simulink model "ForwardKinematic_YuMi"  (R2024a)
(part 16 of 23)

Jacobian_right = [(45469976576263333420024314314012801327919322690514472994826407768302665883518778378566397061146074233600072400531729144381613193100703*cos(q1R))/14196068833898572081041480622812588561594557825924180864872855452746861095964803189964668959253194639858643000122386287764347688058880000 + (975695490161691334754993201031873422779992507225204606318647386416514578573291323958060306800265973057287823586614606841372311747139967*sin(q1R))/56784275335594288324165922491250354246378231303696723459491421810987444383859212759858675837012778559434572000489545151057390752235520000 + (27*cos(q5R)*((7514214926474921*sin(q4R)*((9007199067919185*cos(q3R)*((23235800371559029388956996013805*cos(q1R))/40564819207303340847894502572032 - (17274190877287359225804725738355*sin(q1R))/162259276829213363391578010288128))/9007199254740992 + (7514214926474921*cos(q3R)*((7514214926474921*cos(q2R)*((2579692110316253*cos(q1R))/4503599627370496 - (1917820484151683*sin(q1R))/18014398509481984))/36893488147419103232 + sin(q2R)*((1917820484151683*cos(q1R))/18014398509481984 + (2579692110316253*sin(q1R))/4503599627370496)))/36893488147419103232 - sin(q3R)*(cos(q2R)*((1917820484151683*cos(q1R))/18014398509481984 + (2579692110316253*sin(q1R))/4503599627370496) - (7514214926474921*sin(q2R)*((2579692110316253*cos(q1R))/4503599627370496 - (1917820484151683*sin(q1R))/18014398509481984))/36893488147419103232)))/36893488147419103232 + ((9007199067919185*cos(q4R))/9007199254740992 - (234819211581865*sin(q4R))/1152921504606846976)*((129801982932889585091297864435361917839115294955*sin(q1R))/5986310706507378352962293074805895248510699696029696 - (174598797980560374072834504815488878557302284405*cos(q1R))/1496577676626844588240573268701473812127674924007424 + (67682029681889335677290557259385*cos(q2R)*((2579692110316253*cos(q1R))/4503599627370496 - (1917820484151683*sin(q1R))/18014398509481984))/332306998946228968225951765070086144 + (9007199067919185*sin(q2R)*((1917820484151683*cos(q1R))/18014398509481984 + (2579692110316253*sin(q1R))/4503599627370496))/9007199254740992) + ((7514214926474921*cos(q4R))/36893488147419103232 + (4503599440548691*sin(q4R))/4503599627370496)*((9007199067919185*sin(q3R)*((23235800371559029388956996013805*cos(q1R))/40564819207303340847894502572032 - (17274190877287359225804725738355*sin(q1R))/162259276829213363391578010288128))/9007199254740992 + cos(q3R)*(cos(q2R)*((1917820484151683*cos(q1R))/18014398509481984 + (2579692110316253*sin(q1R))/4503599627370496) - (7514214926474921*sin(q2R)*((2579692110316253*cos(q1R))/4503599627370496 - (1917820484151683*sin(q1R))/18014398509481984))/36893488147419103232) + (7514214926474921*sin(q3R)*((7514214926474921*cos(q2R)*((2579692110316253*cos(q1R))/4503599627370496 - (1917820484151683*sin(q1R))/18014398509481984))/36893488147419103232 + sin(q2R)*((1917820484151683*cos(q1R))/18014398509481984 + (2579692110316253*sin(q1R))/4503599627370496)))/36893488147419103232)))/1000 - (202883803014822867*sin(q5R)*((7514214926474921*cos(q4R)*((9007199067919185*cos(q3R)*((23235800371559029388956996013805*cos(q1R))/40564819207303340847894502572032 - (17274190877287359225804725738355*sin(q1R))/162259276829213363391578010288128))/9007199254740992 + (7514214926474921*cos(q3R)*((7514214926474921*cos(q2R)*((2579692110316253*cos(q1R))/4503599627370496 - (1917820484151683*sin(q1R))/18014398509481984))/36893488147419103232 + sin(q2R)*((1917820484151683*cos(q1R))/18014398509481984 + (2579692110316253*sin(q1R))/4503599627370496)))/36893488147419103232 - sin(q3R)*(cos(q2R)*((1917820484151683*cos(q1R))/18014398509481984 + (2579692110316253*sin(q1R))/4503599627370496) - (7514214926474921*sin(q2R)*((2579692110316253*cos(q1R))/4503599627370496 - (1917820484151683*sin(q1R))/18014398509481984))/36893488147419103232)))/36893488147419103232 - ((234819211581865*cos(q4R))/1152921504606846976 + (9007199067919185*sin(q4R))/9007199254740992)*((129801982932889585091297864435361917839115294955*sin(q1R))/5986310706507378352962293074805895248510699696029696 - (174598797980560374072834504815488878557302284405*cos(q1R))/1496577676626844588240573268701473812127674924007424 + (67682029681889335677290557259385*cos(q2R)*((2579692110316253*cos(q1R))/4503599627370496 - (1917820484151683*sin(q1R))/18014398509481984))/332306998946228968225951765070086144 + (9007199067919185*sin(q2R)*((1917820484151683*cos(q1R))/18014398509481984 + (2579692110316253*sin(q1R))/4503599627370496))/9007199254740992) + ((4503599440548691*cos(q4R))/4503599627370496 - (7514214926474921*sin(q4R))/36893488147419103232)*((9007199067919185*sin(q3R)*((23235800371559029388956996013805*cos(q1R))/40564819207303340847894502572032 - (17274190877287359225804725738355*sin(q1R))/162259276829213363391578010288128))/9007199254740992 + cos(q3R)*(cos(q2R)*((1917820484151683*cos(q1R))/18014398509481984 + (2579692110316253*sin(q1R))/4503599627370496) - (7514214926474921*sin(q2R)*((2579692110316253*cos(q1R))/4503599627370496 - (1917820484151683*sin(q1R))/18014398509481984))/36893488147419103232) + (7514214926474921*sin(q3R)*((7514214926474921*cos(q2R)*((2579692110316253*cos(q1R))/4503599627370496 - (1917820484151683*sin(q1R))/18014398509481984))/36893488147419103232 + sin(q2R)*((1917820484151683*cos(q1R))/18014398509481984 + (2579692110316253*sin(q1R))/4503599627370496)))/36893488147419103232)))/36893488147419103232000 - (610321541873521657855151997354401418608858870661075444886782706002880706727*cos(q4R)*((9007199067919185*cos(q3R)*((23235800371559029388956996013805*cos(q1R))/40564819207303340847894502572032 - (17274190877287359225804725738355*sin(q1R))/162259276829213363391578010288128))/9007199254740992 + (7514214926474921*cos(q3R)*((7514214926474921*cos(q2R)*((2579692110316253*cos(q1R))/4503599627370496 - (1917820484151683*sin(q1R))/18014398509481984))/36893488147419103232 + sin(q2R)*((1917820484151683*cos(q1R))/18014398509481984 + (2579692110316253*sin(q1R))/4503599627370496)))/36893488147419103232 - sin(q3R)*(cos(q2R)*((1917820484151683*cos(q1R))/18014398509481984 + (2579692110316253*sin(q1R))/4503599627370496) - (7514214926474921*sin(q2R)*((2579692110316253*cos(q1R))/4503599627370496 - (1917820484151683*sin(q1R))/18014398509481984))/36893488147419103232)))/11307821214581659709333104004754678501295896940003961331978279688272766566400000 - (584133382113593486367040631332731*cos(q6R)*((2056090974134078155817856050893176283501835309672875224633265471054954772650875*cos(q1R))/2085924839766513752338888384931203236916703635113918720651407820138886450957656787131798913024 - (1528559695827542654859482295756575375660057523072748460051910118126597762297125*sin(q1R))/8343699359066055009355553539724812947666814540455674882605631280555545803830627148527195652096 + (67682029681889335677290557259385*cos(q4R)*((9007199067919185*cos(q3R)*((23235800371559029388956996013805*cos(q1R))/40564819207303340847894502572032 - (17274190877287359225804725738355*sin(q1R))/162259276829213363391578010288128))/9007199254740992 + (7514214926474921*cos(q3R)*((7514214926474921*cos(q2R)*((2579692110316253*cos(q1R))/4503599627370496 - (1917820484151683*sin(q1R))/18014398509481984))/36893488147419103232 + sin(q2R)*((1917820484151683*cos(q1R))/18014398509481984 + (2579692110316253*sin(q1R))/4503599627370496)))/36893488147419103232 - sin(q3R)*(cos(q2R)*((1917820484151683*cos(q1R))/18014398509481984 + (2579692110316253*sin(q1R))/4503599627370496) - (7514214926474921*sin(q2R)*((2579692110316253*cos(q1R))/4503599627370496 - (1917820484151683*sin(q1R))/18014398509481984))/36893488147419103232)))/332306998946228968225951765070086144 - (9007199067919185*((234819211581865*cos(q4R))/1152921504606846976 + (9007199067919185*sin(q4R))/9007199254740992)*((129801982932889585091297864435361917839115294955*sin(q1R))/5986310706507378352962293074805895248510699696029696 - (174598797980560374072834504815488878557302284405*cos(q1R))/1496577676626844588240573268701473812127674924007424 + (67682029681889335677290557259385*cos(q2R)*((2579692110316253*cos(q1R))/4503599627370496 - (1917820484151683*sin(q1R))/18014398509481984))/332306998946228968225951765070086144 + (9007199067919185*sin(q2R)*((1917820484151683*cos(q1R))/18014398509481984 + (2579692110316253*sin(q1R))/4503599627370496))/9007199254740992))/9007199254740992 - (609625514665592237562888769449172969868262801225*cos(q3R)*((23235800371559029388956996013805*cos(q1R))/40564819207303340847894502572032 - (17274190877287359225804725738355*sin(q1R))/162259276829213363391578010288128))/2993155353253689176481146537402947624255349848014848 + (15893040848161638993908057577265778144967053025*sin(q3R)*((23235800371559029388956996013805*cos(q1R))/40564819207303340847894502572032 - (17274190877287359225804725738355*sin(q1R))/162259276829213363391578010288128))/383123885216472214589586756787577295904684780545900544 + (9007199067919185*((4503599440548691*cos(q4R))/4503599627370496 - (7514214926474921*sin(q4R))/36893488147419103232)*((9007199067919185*sin(q3R)*((23235800371559029388956996013805*cos(q1R))/40564819207303340847894502572032 - (17274190877287359225804725738355*sin(q1R))/162259276829213363391578010288128))/9007199254740992 + cos(q3R)*(cos(q2R)*((1917820484151683*cos(q1R))/18014398509481984 + (2579692110316253*sin(q1R))/4503599627370496) - (7514214926474921*sin(q2R)*((2579692110316253*cos(q1R))/4503599627370496 - (1917820484151683*sin(q1R))/18014398509481984))/36893488147419103232) + (7514214926474921*sin(q3R)*((7514214926474921*cos(q2R)*((2579692110316253*cos(q1R))/4503599627370496 - (1917820484151683*sin(q1R))/18014398509481984))/36893488147419103232 + sin(q2R)*((1917820484151683*cos(q1R))/18014398509481984 + (2579692110316253*sin(q1R))/4503599627370496)))/36893488147419103232))/9007199254740992 + (1764482024691522628700660907665*cos(q3R)*(cos(q2R)*((1917820484151683*cos(q1R))/18014398509481984 + (2579692110316253*sin(q1R))/4503599627370496) - (7514214926474921*sin(q2R)*((2579692110316253*cos(q1R))/4503599627370496 - (1917820484151683*sin(q1R))/18014398509481984))/36893488147419103232))/42535295865117307932921825928971026432 - (508577317689771495245073589786522929324694383585*cos(q3R)*((7514214926474921*cos(q2R)*((2579692110316253*cos(q1R))/4503599627370496 - (1917820484151683*sin(q1R))/18014398509481984))/36893488147419103232 + sin(q2R)*((1917820484151683*cos(q1R))/18014398509481984 + (2579692110316253*sin(q1R))/4503599627370496)))/12259964326927110866866776217202473468949912977468817408 + (67682029681889335677290557259385*sin(q3R)*(cos(q2R)*((1917820484151683*cos(q1R))/18014398509481984 + (2579692110316253*sin(q1R))/4503599627370496) - (7514214926474921*sin(q2R)*((2579692110316253*cos(q1R))/4503599627370496 - (1917820484151683*sin(q1R))/18014398509481984))/36893488147419103232))/332306998946228968225951765070086144 + (13258697167433729449897784796786197386719169465*sin(q3R)*((7514214926474921*cos(q2R)*((2579692110316253*cos(q1R))/4503599627370496 - (1917820484151683*sin(q1R))/18014398509481984))/36893488147419103232 + sin(q2R)*((1917820484151683*cos(q1R))/18014398509481984 + (2579692110316253*sin(q1R))/4503599627370496)))/1569275433846670190958947355801916604025588861116008628224 - (797029601289130257223357069404502671534492977261568326111352375*cos(q2R)*((2579692110316253*cos(q1R))/4503599627370496 - (1917820484151683*sin(q1R))/18014398509481984))/463168356949264781694283940034751631413079938662562256157830336031652518559744 - (106069577339469832923929692356850887620017617375*sin(q2R)*((1917820484151683*cos(q1R))/18014398509481984 + (2579692110316253*sin(q1R))/4503599627370496))/12554203470773361527671578846415332832204710888928069025792))/16225927682921336339157801028812800 + (94754841554645069948206780163139*sin(q5R)*((7514214926474921*sin(q4R)*((9007199067919185*cos(q3R)*((23235800371559029388956996013805*cos(q1R))/40564819207303340847894502572032 - (17274190877287359225804725738355*sin(q1R))/162259276829213363391578010288128))/9007199254740992 + (7514214926474921*cos(q3R)*((7514214926474921*cos(q2R)*((2579692110316253*cos(q1R))/4503599627370496 - (1917820484151683*sin(q1R))/18014398509481984))/36893488147419103232 + sin(q2R)*((1917820484151683*cos(q1R))/18014398509481984 + (2579692110316253*sin(q1R))/4503599627370496)))/36893488147419103232 - sin(q3R)*(cos(q2R)*((1917820484151683*cos(q1R))/18014398509481984 + (2579692110316253*sin(q1R))/4503599627370496) - (7514214926474921*sin(q2R)*((2579692110316253*cos(q1R))/4503599627370496 - (1917820484151683*sin(q1R))/18014398509481984))/36893488147419103232)))/36893488147419103232 + ((9007199067919185*cos(q4R))/9007199254740992 - (234819211581865*sin(q4R))/1152921504606846976)*((129801982932889585091297864435361917839115294955*sin(q1R))/5986310706507378352962293074805895248510699696029696 - (174598797980560374072834504815488878557302284405*cos(q1R))/1496577676626844588240573268701473812127674924007424 + (67682029681889335677290557259385*cos(q2R)*((2579692110316253*cos(q1R))/4503599627370496 - (1917820484151683*sin(q1R))/18014398509481984))/332306998946228968225951765070086144 + (9007199067919185*sin(q2R)*((1917820484151683*cos(q1R))/18014398509481984 + (2579692110316253*sin(q1R))/4503599627370496))/9007199254740992) + ((7514214926474921*cos(q4R))/36893488147419103232 + (4503599440548691*sin(q4R))/4503599627370496)*((9007199067919185*sin(q3R)*((23235800371559029388956996013805*cos(q1R))/40564819207303340847894502572032 - (17274190877287359225804725738355*sin(q1R))/162259276829213363391578010288128))/9007199254740992 + cos(q3R)*(cos(q2R)*((1917820484151683*cos(q1R))/18014398509481984 + (2579692110316253*sin(q1R))/4503599627370496) - (7514214926474921*sin(q2R)*((2579692110316253*cos(q1R))/4503599627370496 - (1917820484151683*sin(q1R))/18014398509481984))/36893488147419103232) + (7514214926474921*sin(q3R)*((7514214926474921*cos(q2R)*((2579692110316253*cos(q1R))/4503599627370496 - (1917820484151683*sin(q1R))/18014398509481984))/36893488147419103232 + sin(q2R)*((1917820484151683*cos(q1R))/18014398509481984 + (2579692110316253*sin(q1R))/4503599627370496)))/36893488147419103232)))/66461399789245793645190353014017228800 - (608651409044468601*sin(q4R)*((9007199067919185*cos(q3R)*((23235800371559029388956996013805*cos(q1R))/40564819207303340847894502572032 - (17274190877287359225804725738355*sin(q1R))/162259276829213363391578010288128))/9007199254740992 + (7514214926474921*cos(q3R)*((7514214926474921*cos(q2R)*((2579692110316253*cos(q1R))/4503599627370496 - (1917820484151683*sin(q1R))/18014398509481984))/36893488147419103232 + sin(q2R)*((1917820484151683*cos(q1R))/18014398509481984 + (2579692110316253*sin(q1R))/4503599627370496)))/36893488147419103232 - sin(q3R)*(cos(q2R)*((1917820484151683*cos(q1R))/18014398509481984 + (2579692110316253*sin(q1R))/4503599627370496) - (7514214926474921*sin(q2R)*((2579692110316253*cos(q1R))/4503599627370496 - (1917820484151683*sin(q1R))/18014398509481984))/36893488147419103232)))/73786976294838206464000 - (48638874966763599*sin(q6R)*((2056090974134078155817856050893176283501835309672875224633265471054954772650875*cos(q1R))/2085924839766513752338888384931203236916703635113918720651407820138886450957656787131798913024 - (1528559695827542654859482295756575375660057523072748460051910118126597762297125*sin(q1R))/8343699359066055009355553539724812947666814540455674882605631280555545803830627148527195652096 + (67682029681889335677290557259385*cos(q4R)*((9007199067919185*cos(q3R)*((23235800371559029388956996013805*cos(q1R))/40564819207303340847894502572032 - (17274190877287359225804725738355*sin(q1R))/162259276829213363391578010288128))/9007199254740992 + (7514214926474921*cos(q3R)*((7514214926474921*cos(q2R)*((2579692110316253*cos(q1R))/4503599627370496 - (1917820484151683*sin(q1R))/18014398509481984))/36893488147419103232 + sin(q2R)*((1917820484151683*cos(q1R))/18014398509481984 + (2579692110316253*sin(q1R))/4503599627370496)))/36893488147419103232 - sin(q3R)*(cos(q2R)*((1917820484151683*cos(q1R))/18014398509481984 + (2579692110316253*sin(q1R))/4503599627370496) - (7514214926474921*sin(q2R)*((2579692110316253*cos(q1R))/4503599627370496 - (1917820484151683*sin(q1R))/18014398509481984))/36893488147419103232)))/332306998946228968225951765070086144 - (9007199067919185*((234819211581865*cos(q4R))/1152921504606846976 + (9007199067919185*sin(q4R))/9007199254740992)*((129801982932889585091297864435361917839115294955*sin(q1R))/5986310706507378352962293074805895248510699696029696 - (174598797980560374072834504815488878557302284405*cos(q1R))/1496577676626844588240573268701473812127674924007424 + (67682029681889335677290557259385*cos(q2R)*((2579692110316253*cos(q1R))/4503599627370496 - (1917820484151683*sin(q1R))/18014398509481984))/332306998946228968225951765070086144 + (9007199067919185*sin(q2R)*((1917820484151683*cos(q1R))/18014398509481984 + (2579692110316253*sin(q1R))/4503599627370496))/9007199254740992))/9007199254740992 - (609625514665592237562888769449172969868262801225*cos(q3R)*((23235800371559029388956996013805*cos(q1R))/40564819207303340847894502572032 - (17274190877287359225804725738355*sin(q1R))/162259276829213363391578010288128))/2993155353253689176481146537402947624255349848014848 + (15893040848161638993908057577265778144967053025*sin(q3R)*((23235800371559029388956996013805*cos(q1R))/40564819207303340847894502572032 - (17274190877287359225804725738355*sin(q1R))/162259276829213363391578010288128))/383123885216472214589586756787577295904684780545900544 + (9007199067919185*((4503599440548691*cos(q4R))/4503599627370496 - (7514214926474921*sin(q4R))/36893488147419103232)*((9007199067919185*sin(q3R)*((23235800371559029388956996013805*cos(q1R))/40564819207303340847894502572032 - (17274190877287359225804725738355*sin(q1R))/162259276829213363391578010288128))/9007199254740992 + cos(q3R)*(cos(q2R)*((1917820484151683*cos(q1R))/18014398509481984 + (2579692110316253*sin(q1R))/4503599627370496) - (7514214926474921*sin(q2R)*((2579692110316253*cos(q1R))/4503599627370496 - (1917820484151683*sin(q1R))/18014398509481984))/36893488147419103232) + (7514214926474921*sin(q3R)*((7514214926474921*cos(q2R)*((2579692110316253*cos(q1R))/4503599627370496 - (1917820484151683*sin(q1R))/18014398509481984))/36893488147419103232 + sin(q2R)*((1917820484151683*cos(q1R))/18014398509481984 + (2579692110316253*sin(q1R))/4503599627370496)))/36893488147419103232))/9007199254740992 + (1764482024691522628700660907665*cos(q3R)*(cos(q2R)*((1917820484151683*cos(q1R))/18014398509481984 + (2579692110316253*sin(q1R))/4503599627370496) - (7514214926474921*sin(q2R)*((2579692110316253*cos(q1R))/4503599627370496 - (1917820484151683*sin(q1R))/18014398509481984))/36893488147419103232))/42535295865117307932921825928971026432 - (508577317689771495245073589786522929324694383585*cos(q3R)*((7514214926474921*cos(q2R)*((2579692110316253*cos(q1R))/4503599627370496 - (1917820484151683*sin(q1R))/18014398509481984))/36893488147419103232 + sin(q2R)*((1917820484151683*cos(q1R))/18014398509481984 + (2579692110316253*sin(q1R))/4503599627370496)))/12259964326927110866866776217202473468949912977468817408 + (67682029681889335677290557259385*sin(q3R)*(cos(q2R)*((1917820484151683*cos(q1R))/18014398509481984 + (2579692110316253*sin(q1R))/4503599627370496) - (7514214926474921*sin(q2R)*((2579692110316253*cos(q1R))/4503599627370496 - (1917820484151683*sin(q1R))/18014398509481984))/36893488147419103232))/332306998946228968225951765070086144 + (13258697167433729449897784796786197386719169465*sin(q3R)*((7514214926474921*cos(q2R)*((2579692110316253*cos(q1R))/4503599627370496 - (1917820484151683*sin(q1R))/18014398509481984))/36893488147419103232 + sin(q2R)*((1917820484151683*cos(q1R))/18014398509481984 + (2579692110316253*sin(q1R))/4503599627370496)))/1569275433846670190958947355801916604025588861116008628224 - (797029601289130257223357069404502671534492977261568326111352375*cos(q2R)*((2579692110316253*cos(q1R))/4503599627370496 - (1917820484151683*sin(q1R))/18014398509481984))/463168356949264781694283940034751631413079938662562256157830336031652518559744 - (106069577339469832923929692356850887620017617375*sin(q2R)*((1917820484151683*cos(q1R))/18014398509481984 + (2579692110316253*sin(q1R))/4503599627370496))/12554203470773361527671578846415332832204710888928069025792))/1801439850948198400 - (81*((9007199067919185*cos(q4R))/9007199254740992 - (234819211581865*sin(q4R))/1152921504606846976)*((129801982932889585091297864435361917839115294955*sin(q1R))/5986310706507378352962293074805895248510699696029696 - (174598797980560374072834504815488878557302284405*cos(q1R))/1496577676626844588240573268701473812127674924007424 + (67682029681889335677290557259385*cos(q2R)*((2579692110316253*cos(q1R))/4503599627370496 - (1917820484151683*sin(q1R))/18014398509481984))/332306998946228968225951765070086144 + (9007199067919185*sin(q2R)*((1917820484151683*cos(q1R))/18014398509481984 + (2579692110316253*sin(q1R))/4503599627370496))/9007199254740992))/2000 + (81222263116692158804177042061221826384594597321566869716687*((234819211581865*cos(q4R))/1152921504606846976 + (9007199067919185*sin(q4R))/9007199254740992)*((129801982932889585091297864435361917839115294955*sin(q1R))/5986310706507378352962293074805895248510699696029696 - (174598797980560374072834504815488878557302284405*cos(q1R))/1496577676626844588240573268701473812127674924007424 + (67682029681889335677290557259385*cos(q2R)*((2579692110316253*cos(q1R))/4503599627370496 - (1917820484151683*sin(q1R))/18014398509481984))/332306998946228968225951765070086144 + (9007199067919185*sin(q2R)*((1917820484151683*cos(q1R))/18014398509481984 + (2579692110316253*sin(q1R))/4503599627370496))/9007199254740992))/306499108173177771671669405430061836723747824436720435200000 - (170695144106365826517608855445768431563113584343*cos(q5R)*((273626851807209941619219010639387076236787289365779842797695875*cos(q1R))/56539106072908298546665520023773392506479484700019806659891398441363832832 - (203422408166946418981152780445187297537016008229516441756292125*sin(q1R))/226156424291633194186662080095093570025917938800079226639565593765455331328 - (81129635049124235038645691064225*cos(q3R)*((23235800371559029388956996013805*cos(q1R))/40564819207303340847894502572032 - (17274190877287359225804725738355*sin(q1R))/162259276829213363391578010288128))/81129638414606681695789005144064 + (2115063383689692319117831580025*sin(q3R)*((23235800371559029388956996013805*cos(q1R))/40564819207303340847894502572032 - (17274190877287359225804725738355*sin(q1R))/162259276829213363391578010288128))/10384593717069655257060992658440192 + (234819211581865*cos(q3R)*(cos(q2R)*((1917820484151683*cos(q1R))/18014398509481984 + (2579692110316253*sin(q1R))/4503599627370496) - (7514214926474921*sin(q2R)*((2579692110316253*cos(q1R))/4503599627370496 - (1917820484151683*sin(q1R))/18014398509481984))/36893488147419103232))/1152921504606846976 - (67682029681889335677290557259385*cos(q3R)*((7514214926474921*cos(q2R)*((2579692110316253*cos(q1R))/4503599627370496 - (1917820484151683*sin(q1R))/18014398509481984))/36893488147419103232 + sin(q2R)*((1917820484151683*cos(q1R))/18014398509481984 + (2579692110316253*sin(q1R))/4503599627370496)))/332306998946228968225951765070086144 + (9007199067919185*sin(q3R)*(cos(q2R)*((1917820484151683*cos(q1R))/18014398509481984 + (2579692110316253*sin(q1R))/4503599627370496) - (7514214926474921*sin(q2R)*((2579692110316253*cos(q1R))/4503599627370496 - (1917820484151683*sin(q1R))/18014398509481984))/36893488147419103232))/9007199254740992 + (1764482024691522628700660907665*sin(q3R)*((7514214926474921*cos(q2R)*((2579692110316253*cos(q1R))/4503599627370496 - (1917820484151683*sin(q1R))/18014398509481984))/36893488147419103232 + sin(q2R)*((1917820484151683*cos(q1R))/18014398509481984 + (2579692110316253*sin(q1R))/4503599627370496)))/42535295865117307932921825928971026432 - (106069577339469832923929692356850887620017617375*cos(q2R)*((2579692110316253*cos(q1R))/4503599627370496 - (1917820484151683*sin(q1R))/18014398509481984))/12554203470773361527671578846415332832204710888928069025792 - (14115856197532180673579726082375*sin(q2R)*((1917820484151683*cos(q1R))/18014398509481984 + (2579692110316253*sin(q1R))/4503599627370496))/340282366920938463463374607431768211456))/119726214130147567059245861496117904970213993920593920 + (48638874966763599*sin(q5R)*((273626851807209941619219010639387076236787289365779842797695875*cos(q1R))/56539106072908298546665520023773392506479484700019806659891398441363832832 - (203422408166946418981152780445187297537016008229516441756292125*sin(q1R))/226156424291633194186662080095093570025917938800079226639565593765455331328 - (81129635049124235038645691064225*cos(q3R)*((23235800371559029388956996013805*cos(q1R))/40564819207303340847894502572032 - (17274190877287359225804725738355*sin(q1R))/162259276829213363391578010288128))/81129638414606681695789005144064 + (2115063383689692319117831580025*sin(q3R)*((23235800371559029388956996013805*cos(q1R))/40564819207303340847894502572032 - (17274190877287359225804725738355*sin(q1R))/162259276829213363391578010288128))/10384593717069655257060992658440192 + (234819211581865*cos(q3R)*(cos(q2R)*((1917820484151683*cos(q1R))/18014398509481984 + (2579692110316253*sin(q1R))/4503599627370496) - (7514214926474921*sin(q2R)*((2579692110316253*cos(q1R))/4503599627370496 - (1917820484151683*sin(q1R))/18014398509481984))/36893488147419103232))/1152921504606846976 - (67682029681889335677290557259385*cos(q3R)*((7514214926474921*cos(q2R)*((2579692110316253*cos(q1R))/4503599627370496 - (1917820484151683*sin(q1R))/18014398509481984))/36893488147419103232 + sin(q2R)*((1917820484151683*cos(q1R))/18014398509481984 + (2579692110316253*sin(q1R))/4503599627370496)))/332306998946228968225951765070086144 + (9007199067919185*sin(q3R)*(cos(q2R)*((1917820484151683*cos(q1R))/18014398509481984 + (2579692110316253*sin(q1R))/4503599627370496) - (7514214926474921*sin(q2R)*((2579692110316253*cos(q1R))/4503599627370496 - (1917820484151683*sin(q1R))/18014398509481984))/36893488147419103232))/9007199254740992 + (1764482024691522628700660907665*sin(q3R)*((7514214926474921*cos(q2R)*((2579692110316253*cos(q1R))/4503599627370496 - (1917820484151683*sin(q1R))/18014398509481984))/36893488147419103232 + sin(q2R)*((1917820484151683*cos(q1R))/18014398509481984 + (2579692110316253*sin(q1R))/4503599627370496)))/42535295865117307932921825928971026432 - (106069577339469832923929692356850887620017617375*cos(q2R)*((2579692110316253*cos(q1R))/4503599627370496 - (1917820484151683*sin(q1R))/18014398509481984))/12554203470773361527671578846415332832204710888928069025792 - (14115856197532180673579726082375*sin(q2R)*((1917820484151683*cos(q1R))/18014398509481984 + (2579692110316253*sin(q1R))/4503599627370496))/340282366920938463463374607431768211456))/1801439850948198400 - (2436553109258773196144549622003023*cos(q6R)*(sin(q5R)*((7514214926474921*sin(q4R)*((9007199067919185*cos(q3R)*((23235800371559029388956996013805*cos(q1R))/40564819207303340847894502572032 - (17274190877287359225804725738355*sin(q1R))/162259276829213363391578010288128))/9007199254740992 + (7514214926474921*cos(q3R)*((7514214926474921*cos(q2R)*((2579692110316253*cos(q1R))/4503599627370496 - (1917820484151683*sin(q1R))/18014398509481984))/36893488147419103232 + sin(q2R)*((1917820484151683*cos(q1R))/18014398509481984 + (2579692110316253*sin(q1R))/4503599627370496)))/36893488147419103232 - sin(q3R)*(cos(q2R)*((1917820484151683*cos(q1R))/18014398509481984 + (2579692110316253*sin(q1R))/4503599627370496) - (7514214926474921*sin(q2R)*((2579692110316253*cos(q1R))/4503599627370496 - (1917820484151683*sin(q1R))/18014398509481984))/36893488147419103232)))/36893488147419103232 + ((9007199067919185*cos(q4R))/9007199254740992 - (234819211581865*sin(q4R))/1152921504606846976)*((129801982932889585091297864435361917839115294955*sin(q1R))/5986310706507378352962293074805895248510699696029696 - (174598797980560374072834504815488878557302284405*cos(q1R))/1496577676626844588240573268701473812127674924007424 + (67682029681889335677290557259385*cos(q2R)*((2579692110316253*cos(q1R))/4503599627370496 - (1917820484151683*sin(q1R))/18014398509481984))/332306998946228968225951765070086144 + (9007199067919185*sin(q2R)*((1917820484151683*cos(q1R))/18014398509481984 + (2579692110316253*sin(q1R))/4503599627370496))/9007199254740992) + ((7514214926474921*cos(q4R))/36893488147419103232 + (4503599440548691*sin(q4R))/4503599627370496)*((9007199067919185*sin(q3R)*((23235800371559029388956996013805*cos(q1R))/40564819207303340847894502572032 - (17274190877287359225804725738355*sin(q1R))/162259276829213363391578010288128))/9007199254740992 + cos(q3R)*(cos(q2R)*((1917820484151683*cos(q1R))/18014398509481984 + (2579692110316253*sin(q1R))/4503599627370496) - (7514214926474921*sin(q2R)*((2579692110316253*cos(q1R))/4503599627370496 - (1917820484151683*sin(q1R))/18014398509481984))/36893488147419103232) + (7514214926474921*sin(q3R)*((7514214926474921*cos(q2R)*((2579692110316253*cos(q1R))/4503599627370496 - (1917820484151683*sin(q1R))/18014398509481984))/36893488147419103232 + sin(q2R)*((1917820484151683*cos(q1R))/18014398509481984 + (2579692110316253*sin(q1R))/4503599627370496)))/36893488147419103232)) - (9007199067919185*cos(q5R)*((273626851807209941619219010639387076236787289365779842797695875*cos(q1R))/56539106072908298546665520023773392506479484700019806659891398441363832832 - (203422408166946418981152780445187297537016008229516441756292125*sin(q1R))/226156424291633194186662080095093570025917938800079226639565593765455331328 - (81129635049124235038645691064225*cos(q3R)*((23235800371559029388956996013805*cos(q1R))/40564819207303340847894502572032 - (17274190877287359225804725738355*sin(q1R))/162259276829213363391578010288128))/81129638414606681695789005144064 + (2115063383689692319117831580025*sin(q3R)*((23235800371559029388956996013805*cos(q1R))/40564819207303340847894502572032 - (17274190877287359225804725738355*sin(q1R))/162259276829213363391578010288128))/10384593717069655257060992658440192 + (234819211581865*cos(q3R)*(cos(q2R)*((1917820484151683*cos(q1R))/18014398509481984 + (2579692110316253*sin(q1R))/4503599627370496) - (7514214926474921*sin(q2R)*((2579692110316253*cos(q1R))/4503599627370496 - (1917820484151683*sin(q1R))/18014398509481984))/36893488147419103232))/1152921504606846976 - (67682029681889335677290557259385*cos(q3R)*((7514214926474921*cos(q2R)*((2579692110316253*cos(q1R))/4503599627370496 - (1917820484151683*sin(q1R))/18014398509481984))/36893488147419103232 + sin(q2R)*((1917820484151683*cos(q1R))/18014398509481984 + (2579692110316253*sin(q1R))/4503599627370496)))/332306998946228968225951765070086144 + (9007199067919185*sin(q3R)*(cos(q2R)*((1917820484151683*cos(q1R))/18014398509481984 + (2579692110316253*sin(q1R))/4503599627370496) - (7514214926474921*sin(q2R)*((2579692110316253*cos(q1R))/4503599627370496 - (1917820484151683*sin(q1R))/18014398509481984))/36893488147419103232))/9007199254740992 + (1764482024691522628700660907665*sin(q3R)*((7514214926474921*cos(q2R)*((2579692110316253*cos(q1R))/4503599627370496 - (1917820484151683*sin(q1R))/18014398509481984))/36893488147419103232 + sin(q2R)*((1917820484151683*cos(q1R))/18014398509481984 + (2579692110316253*sin(q1R))/4503599627370496)))/42535295865117307932921825928971026432 - (106069577339469832923929692356850887620017617375*cos(q2R)*((2579692110316253*cos(q1R))/4503599627370496 - (1917820484151683*sin(q1R))/18014398509481984))/12554203470773361527671578846415332832204710888928069025792 - (14115856197532180673579726082375*sin(q2R)*((1917820484151683*cos(q1R))/18014398509481984 + (2579692110316253*sin(q1R))/4503599627370496))/340282366920938463463374607431768211456))/9007199254740992 + (7514214926474921*cos(q5R)*((7514214926474921*cos(q4R)*((9007199067919185*cos(q3R)*((23235800371559029388956996013805*cos(q1R))/40564819207303340847894502572032 - (17274190877287359225804725738355*sin(q1R))/162259276829213363391578010288128))/9007199254740992 + (7514214926474921*cos(q3R)*((7514214926474921*cos(q2R)*((2579692110316253*cos(q1R))/4503599627370496 - (1917820484151683*sin(q1R))/18014398509481984))/36893488147419103232 + sin(q2R)*((1917820484151683*cos(q1R))/18014398509481984 + (2579692110316253*sin(q1R))/4503599627370496)))/36893488147419103232 - sin(q3R)*(cos(q2R)*((1917820484151683*cos(q1R))/18014398509481984 + (2579692110316253*sin(q1R))/4503599627370496) - (7514214926474921*sin(q2R)*((2579692110316253*cos(q1R))/4503599627370496 - (1917820484151683*sin(q1R))/18014398509481984))/36893488147419103232)))/36893488147419103232 - ((234819211581865*cos(q4R))/1152921504606846976 + (9007199067919185*sin(q4R))/9007199254740992)*((129801982932889585091297864435361917839115294955*sin(q1R))/5986310706507378352962293074805895248510699696029696 - (174598797980560374072834504815488878557302284405*cos(q1R))/1496577676626844588240573268701473812127674924007424 + (67682029681889335677290557259385*cos(q2R)*((2579692110316253*cos(q1R))/4503599627370496 - (1917820484151683*sin(q1R))/18014398509481984))/332306998946228968225951765070086144 + (9007199067919185*sin(q2R)*((1917820484151683*cos(q1R))/18014398509481984 + (2579692110316253*sin(q1R))/4503599627370496))/9007199254740992) + ((4503599440548691*cos(q4R))/4503599627370496 - (7514214926474921*sin(q4R))/36893488147419103232)*((9007199067919185*sin(q3R)*((23235800371559029388956996013805*cos(q1R))/40564819207303340847894502572032 - (17274190877287359225804725738355*sin(q1R))/162259276829213363391578010288128))/9007199254740992 + cos(q3R)*(cos(q2R)*((1917820484151683*cos(q1R))/18014398509481984 + (2579692110316253*sin(q1R))/4503599627370496) - (7514214926474921*sin(q2R)*((2579692110316253*cos(q1R))/4503599627370496 - (1917820484151683*sin(q1R))/18014398509481984))/36893488147419103232) + (7514214926474921*sin(q3R)*((7514214926474921*cos(q2R)*((2579692110316253*cos(q1R))/4503599627370496 - (1917820484151683*sin(q1R))/18014398509481984))/36893488147419103232 + sin(q2R)*((1917820484151683*cos(q1R))/18014398509481984 + (2579692110316253*sin(q1R))/4503599627370496)))/36893488147419103232)))/36893488147419103232))/332306998946228968225951765070086144000 - (27*cos(q6R)*(cos(q5R)*((7514214926474921*sin(q4R)*((9007199067919185*cos(q3R)*((23235800371559029388956996013805*cos(q1R))/40564819207303340847894502572032 - (17274190877287359225804725738355*sin(q1R))/162259276829213363391578010288128))/9007199254740992 + (7514214926474921*cos(q3R)*((7514214926474921*cos(q2R)*((2579692110316253*cos(q1R))/4503599627370496 - (1917820484151683*sin(q1R))/18014398509481984))/36893488147419103232 + sin(q2R)*((1917820484151683*cos(q1R))/18014398509481984 + (2579692110316253*sin(q1R))/4503599627370496)))/36893488147419103232 - sin(q3R)*(cos(q2R)*((1917820484151683*cos(q1R))/18014398509481984 + (2579692110316253*sin(q1R))/4503599627370496) - (7514214926474921*sin(q2R)*((2579692110316253*cos(q1R))/4503599627370496 - (1917820484151683*sin(q1R))/18014398509481984))/36893488147419103232)))/36893488147419103232 + ((9007199067919185*cos(q4R))/9007199254740992 - (234819211581865*sin(q4R))/1152921504606846976)*((129801982932889585091297864435361917839115294955*sin(q1R))/5986310706507378352962293074805895248510699696029696 - (174598797980560374072834504815488878557302284405*cos(q1R))/1496577676626844588240573268701473812127674924007424 + (67682029681889335677290557259385*cos(q2R)*((2579692110316253*cos(q1R))/4503599627370496 - (1917820484151683*sin(q1R))/18014398509481984))/332306998946228968225951765070086144 + (9007199067919185*sin(q2R)*((1917820484151683*cos(q1R))/18014398509481984 + (2579692110316253*sin(q1R))/4503599627370496))/9007199254740992) + ((7514214926474921*cos(q4R))/36893488147419103232 + (4503599440548691*sin(q4R))/4503599627370496)*((9007199067919185*sin(q3R)*((23235800371559029388956996013805*cos(q1R))/40564819207303340847894502572032 - (17274190877287359225804725738355*sin(q1R))/162259276829213363391578010288128))/9007199254740992 + cos(q3R)*(cos(q2R)*((1917820484151683*cos(q1R))/18014398509481984 + (2579692110316253*sin(q1R))/4503599627370496) - (7514214926474921*sin(q2R)*((2579692110316253*cos(q1R))/4503599627370496 - (1917820484151683*sin(q1R))/18014398509481984))/36893488147419103232) + (7514214926474921*sin(q3R)*((7514214926474921*cos(q2R)*((2579692110316253*cos(q1R))/4503599627370496 - (1917820484151683*sin(q1R))/18014398509481984))/36893488147419103232 + sin(q2R)*((1917820484151683*cos(q1R))/18014398509481984 + (2579692110316253*sin(q1R))/4503599627370496)))/36893488147419103232)) - (7514214926474921*sin(q5R)*((7514214926474921*cos(q4R)*((9007199067919185*cos(q3R)*((23235800371559029388956996013805*cos(q1R))/40564819207303340847894502572032 - (17274190877287359225804725738355*sin(q1R))/162259276829213363391578010288128))/9007199254740992 + (7514214926474921*cos(q3R)*((7514214926474921*cos(q2R)*((2579692110316253*cos(q1R))/4503599627370496 - (1917820484151683*sin(q1R))/18014398509481984))/36893488147419103232 + sin(q2R)*((1917820484151683*cos(q1R))/18014398509481984 + (2579692110316253*sin(q1R))/4503599627370496)))/36893488147419103232 - sin(q3R)*(cos(q2R)*((1917820484151683*cos(q1R))/18014398509481984 + (2579692110316253*sin(q1R))/4503599627370496) - (7514214926474921*sin(q2R)*((2579692110316253*cos(q1R))/4503599627370496 - (1917820484151683*sin(q1R))/18014398509481984))/36893488147419103232)))/36893488147419103232 - ((234819211581865*cos(q4R))/1152921504606846976 + (9007199067919185*sin(q4R))/9007199254740992)*((129801982932889585091297864435361917839115294955*sin(q1R))/5986310706507378352962293074805895248510699696029696 - (174598797980560374072834504815488878557302284405*cos(q1R))/1496577676626844588240573268701473812127674924007424 + (67682029681889335677290557259385*cos(q2R)*((2579692110316253*cos(q1R))/4503599627370496 - (1917820484151683*sin(q1R))/18014398509481984))/332306998946228968225951765070086144 + (9007199067919185*sin(q2R)*((1917820484151683*cos(q1R))/18014398509481984 + (2579692110316253*sin(q1R))/4503599627370496))/9007199254740992) + ((4503599440548691*cos(q4R))/4503599627370496 - (7514214926474921*sin(q4R))/36893488147419103232)*((9007199067919185*sin(q3R)*((23235800371559029388956996013805*cos(q1R))/40564819207303340847894502572032 - (17274190877287359225804725738355*sin(q1R))/162259276829213363391578010288128))/9007199254740992 + cos(q3R)*(cos(q2R)*((1917820484151683*cos(q1R))/18014398509481984 + (2579692110316253*sin(q1R))/4503599627370496) - (7514214926474921*sin(q2R)*((2579692110316253*cos(q1R))/4503599627370496 - (1917820484151683*sin(q1R))/18014398509481984))/36893488147419103232) + (7514214926474921*sin(q3R)*((7514214926474921*cos(q2R)*((2579692110316253*cos(q1R))/4503599627370496 - (1917820484151683*sin(q1R))/18014398509481984))/36893488147419103232 + sin(q2R)*((1917820484151683*cos(q1R))/18014398509481984 + (2579692110316253*sin(q1R))/4503599627370496)))/36893488147419103232)))/36893488147419103232 + (9007199067919185*sin(q5R)*((273626851807209941619219010639387076236787289365779842797695875*cos(q1R))/56539106072908298546665520023773392506479484700019806659891398441363832832 - (203422408166946418981152780445187297537016008229516441756292125*sin(q1R))/226156424291633194186662080095093570025917938800079226639565593765455331328 - (81129635049124235038645691064225*cos(q3R)*((23235800371559029388956996013805*cos(q1R))/40564819207303340847894502572032 - (17274190877287359225804725738355*sin(q1R))/162259276829213363391578010288128))/81129638414606681695789005144064 + (2115063383689692319117831580025*sin(q3R)*((23235800371559029388956996013805*cos(q1R))/40564819207303340847894502572032 - (17274190877287359225804725738355*sin(q1R))/162259276829213363391578010288128))/10384593717069655257060992658440192 + (234819211581865*cos(q3R)*(cos(q2R)*((1917820484151683*cos(q1R))/18014398509481984 + (2579692110316253*sin(q1R))/4503599627370496) - (7514214926474921*sin(q2R)*((2579692110316253*cos(q1R))/4503599627370496 - (1917820484151683*sin(q1R))/18014398509481984))/36893488147419103232))/1152921504606846976 - (67682029681889335677290557259385*cos(q3R)*((7514214926474921*cos(q2R)*((2579692110316253*cos(q1R))/4503599627370496 - (1917820484151683*sin(q1R))/18014398509481984))/36893488147419103232 + sin(q2R)*((1917820484151683*cos(q1R))/18014398509481984 + (2579692110316253*sin(q1R))/4503599627370496)))/332306998946228968225951765070086144 + (9007199067919185*sin(q3R)*(cos(q2R)*((1917820484151683*cos(q1R))/18014398509481984 + (2579692110316253*sin(q1R))/4503599627370496) - (7514214926474921*sin(q2R)*((2579692110316253*cos(q1R))/4503599627370496 - (1917820484151683*sin(q1R))/18014398509481984))/36893488147419103232))/9007199254740992 + (1764482024691522628700660907665*sin(q3R)*((7514214926474921*cos(q2R)*((2579692110316253*cos(q1R))/4503599627370496 - (1917820484151683*sin(q1R))/18014398509481984))/36893488147419103232 + sin(q2R)*((1917820484151683*cos(q1R))/18014398509481984 + (2579692110316253*sin(q1R))/4503599627370496)))/42535295865117307932921825928971026432 - (106069577339469832923929692356850887620017617375*cos(q2R)*((2579692110316253*cos(q1R))/4503599627370496 - (1917820484151683*sin(q1R))/18014398509481984))/12554203470773361527671578846415332832204710888928069025792 - (14115856197532180673579726082375*sin(q2R)*((1917820484151683*cos(q1R))/18014398509481984 + (2579692110316253*sin(q1R))/4503599627370496))/340282366920938463463374607431768211456))/9007199254740992))/1000 - (202883803014822867*sin(q6R)*(sin(q5R)*((7514214926474921*sin(q4R)*((9007199067919185*cos(q3R)*((23235800371559029388956996013805*cos(q1R))/40564819207303340847894502572032 - (17274190877287359225804725738355*sin(q1R))/162259276829213363391578010288128))/9007199254740992 + (7514214926474921*cos(q3R)*((7514214926474921*cos(q2R)*((2579692110316253*cos(q1R))/4503599627370496 - (1917820484151683*sin(q1R))/18014398509481984))/36893488147419103232 + sin(q2R)*((1917820484151683*cos(q1R))/18014398509481984 + (2579692110316253*sin(q1R))/4503599627370496)))/36893488147419103232 - sin(q3R)*(cos(q2R)*((1917820484151683*cos(q1R))/18014398509481984 + (2579692110316253*sin(q1R))/4503599627370496) - (7514214926474921*sin(q2R)*((2579692110316253*cos(q1R))/4503599627370496 - (1917820484151683*sin(q1R))/18014398509481984))/36893488147419103232)))/36893488147419103232 + ((9007199067919185*cos(q4R))/9007199254740992 - (234819211581865*sin(q4R))/1152921504606846976)*((129801982932889585091297864435361917839115294955*sin(q1R))/5986310706507378352962293074805895248510699696029696 - (174598797980560374072834504815488878557302284405*cos(q1R))/1496577676626844588240573268701473812127674924007424 + (67682029681889335677290557259385*cos(q2R)*((2579692110316253*cos(q1R))/4503599627370496 - (1917820484151683*sin(q1R))/18014398509481984))/332306998946228968225951765070086144 + (9007199067919185*sin(q2R)*((1917820484151683*cos(q1R))/18014398509481984 + (2579692110316253*sin(q1R))/4503599627370496))/9007199254740992) + ((7514214926474921*cos(q4R))/36893488147419103232 + (4503599440548691*sin(q4R))/4503599627370496)*((9007199067919185*sin(q3R)*((23235800371559029388956996013805*cos(q1R))/40564819207303340847894502572032 - (17274190877287359225804725738355*sin(q1R))/162259276829213363391578010288128))/9007199254740992 + cos(q3R)*(cos(q2R)*((1917820484151683*cos(q1R))/18014398509481984 + (2579692110316253*sin(q1R))/4503599627370496) - (7514214926474921*sin(q2R)*((2579692110316253*cos(q1R))/4503599627370496 - (1917820484151683*sin(q1R))/18014398509481984))/36893488147419103232) + (7514214926474921*sin(q3R)*((7514214926474921*cos(q2R)*((2579692110316253*cos(q1R))/4503599627370496 - (1917820484151683*sin(q1R))/18014398509481984))/36893488147419103232 + sin(q2R)*((1917820484151683*cos(q1R))/18014398509481984 + (2579692110316253*sin(q1R))/4503599627370496)))/36893488147419103232)) - (9007199067919185*cos(q5R)*((273626851807209941619219010639387076236787289365779842797695875*cos(q1R))/56539106072908298546665520023773392506479484700019806659891398441363832832 - (203422408166946418981152780445187297537016008229516441756292125*sin(q1R))/226156424291633194186662080095093570025917938800079226639565593765455331328 - (81129635049124235038645691064225*cos(q3R)*((23235800371559029388956996013805*cos(q1R))/40564819207303340847894502572032 - (17274190877287359225804725738355*sin(q1R))/162259276829213363391578010288128))/81129638414606681695789005144064 + (2115063383689692319117831580025*sin(q3R)*((23235800371559029388956996013805*cos(q1R))/40564819207303340847894502572032 - (17274190877287359225804725738355*sin(q1R))/162259276829213363391578010288128))/10384593717069655257060992658440192 + (234819211581865*cos(q3R)*(cos(q2R)*((1917820484151683*cos(q1R))/18014398509481984 + (2579692110316253*sin(q1R))/4503599627370496) - (7514214926474921*sin(q2R)*((2579692110316253*cos(q1R))/4503599627370496 - (1917820484151683*sin(q1R))/18014398509481984))/36893488147419103232))/1152921504606846976 - (67682029681889335677290557259385*cos(q3R)*((7514214926474921*cos(q2R)*((2579692110316253*cos(q1R))/4503599627370496 - (1917820484151683*sin(q1R))/18014398509481984))/36893488147419103232 + sin(q2R)*((1917820484151683*cos(q1R))/18014398509481984 + (2579692110316253*sin(q1R))/4503599627370496)))/332306998946228968225951765070086144 + (9007199067919185*sin(q3R)*(cos(q2R)*((1917820484151683*cos(q1R))/18014398509481984 + (2579692110316253*sin(q1R))/4503599627370496) - (7514214926474921*sin(q2R)*((2579692110316253*cos(q1R))/4503599627370496 - (1917820484151683*sin(q1R))/18014398509481984))/36893488147419103232))/9007199254740992 + (1764482024691522628700660907665*sin(q3R)*((7514214926474921*cos(q2R)*((2579692110316253*cos(q1R))/4503599627370496 - (1917820484151683*sin(q1R))/18014398509481984))/36893488147419103232 + sin(q2R)*((1917820484151683*cos(q1R))/18014398509481984 + (2579692110316253*sin(q1R))/4503599627370496)))/42535295865117307932921825928971026432 - (106069577339469832923929692356850887620017617375*cos(q2R)*((2579692110316253*cos(q1R))/4503599627370496 - (1917820484151683*sin(q1R))/18014398509481984))/12554203470773361527671578846415332832204710888928069025792 - (14115856197532180673579726082375*sin(q2R)*((1917820484151683*cos(q1R))/18014398509481984 + (2579692110316253*sin(q1R))/4503599627370496))/340282366920938463463374607431768211456))/9007199254740992 + (7514214926474921*cos(q5R)*((7514214926474921*cos(q4R)*((9007199067919185*cos(q3R)*((23235800371559029388956996013805*cos(q1R))/40564819207303340847894502572032 - (17274190877287359225804725738355*sin(q1R))/162259276829213363391578010288128))/9007199254740992 + (7514214926474921*cos(q3R)*((7514214926474921*cos(q2R)*((2579692110316253*cos(q1R))/4503599627370496 - (1917820484151683*sin(q1R))/18014398509481984))/36893488147419103232 + sin(q2R)*((1917820484151683*cos(q1R))/18014398509481984 + (2579692110316253*sin(q1R))/4503599627370496)))/36893488147419103232 - sin(q3R)*(cos(q2R)*((1917820484151683*cos(q1R))/18014398509481984 + (2579692110316253*sin(q1R))/4503599627370496) - (7514214926474921*sin(q2R)*((2579692110316253*cos(q1R))/4503599627370496 - (1917820484151683*sin(q1R))/18014398509481984))/36893488147419103232)))/36893488147419103232 - ((234819211581865*cos(q4R))/1152921504606846976 + (9007199067919185*sin(q4R))/9007199254740992)*((129801982932889585091297864435361917839115294955*sin(q1R))/5986310706507378352962293074805895248510699696029696 - (174598797980560374072834504815488878557302284405*cos(q1R))/1496577676626844588240573268701473812127674924007424 + (67682029681889335677290557259385*cos(q2R)*((2579692110316253*cos(q1R))/4503599627370496 - (1917820484151683*sin(q1R))/18014398509481984))/332306998946228968225951765070086144 + (9007199067919185*sin(q2R)*((1917820484151683*cos(q1R))/18014398509481984 + (2579692110316253*sin(q1R))/4503599627370496))/9007199254740992) + ((4503599440548691*cos(q4R))/4503599627370496 - (7514214926474921*sin(q4R))/36893488147419103232)*((9007199067919185*sin(q3R)*((23235800371559029388956996013805*cos(q1R))/40564819207303340847894502572032 - (17274190877287359225804725738355*sin(q1R))/162259276829213363391578010288128))/9007199254740992 + cos(q3R)*(cos(q2R)*((1917820484151683*cos(q1R))/18014398509481984 + (2579692110316253*sin(q1R))/4503599627370496) - (7514214926474921*sin(q2R)*((2579692110316253*cos(q1R))/4503599627370496 - (1917820484151683*sin(q1R))/18014398509481984))/36893488147419103232) + (7514214926474921*sin(q3R)*((7514214926474921*cos(q2R)*((2579692110316253*cos(q1R))/4503599627370496 - (1917820484151683*sin(q1R))/18014398509481984))/36893488147419103232 + sin(q2R)*((1917820484151683*cos(q1R))/18014398509481984 + (2579692110316253*sin(q1R))/4503599627370496)))/36893488147419103232)))/36893488147419103232))/36893488147419103232000 + (83301539375654672537075965313343183841442266989297270401707771044036658496661398777306991*cos(q3R)*((23235800371559029388956996013805*cos(q1R))/40564819207303340847894502572032 - (17274190877287359225804725738355*sin(q1R))/162259276829213363391578010288128))/4074071952668972172536891376818756322102936787331872501272280898708762599526673412366794752000 + (324259171862923063*sin(q6R)*(cos(q5R)*((7514214926474921*sin(q4R)*((9007199067919185*cos(q3R)*((23235800371559029388956996013805*cos(q1R))/40564819207303340847894502572032 - (17274190877287359225804725738355*sin(q1R))/162259276829213363391578010288128))/9007199254740992 + (7514214926474921*cos(q3R)*((7514214926474921*cos(q2R)*((2579692110316253*cos(q1R))/4503599627370496 - (1917820484151683*sin(q1R))/18014398509481984))/36893488147419103232 + sin(q2R)*((1917820484151683*cos(q1R))/18014398509481984 + (2579692110316253*sin(q1R))/4503599627370496)))/36893488147419103232 - sin(q3R)*(cos(q2R)*((1917820484151683*cos(q1R))/18014398509481984 + (2579692110316253*sin(q1R))/4503599627370496) - (7514214926474921*sin(q2R)*((2579692110316253*cos(q1R))/4503599627370496 - (1917820484151683*sin(q1R))/18014398509481984))/36893488147419103232)))/36893488147419103232 + ((9007199067919185*cos(q4R))/9007199254740992 - (234819211581865*sin(q4R))/1152921504606846976)*((129801982932889585091297864435361917839115294955*sin(q1R))/5986310706507378352962293074805895248510699696029696 - (174598797980560374072834504815488878557302284405*cos(q1R))/1496577676626844588240573268701473812127674924007424 + (67682029681889335677290557259385*cos(q2R)*((2579692110316253*cos(q1R))/4503599627370496 - (1917820484151683*sin(q1R))/18014398509481984))/332306998946228968225951765070086144 + (9007199067919185*sin(q2R)*((1917820484151683*cos(q1R))/18014398509481984 + (2579692110316253*sin(q1R))/4503599627370496))/9007199254740992) + ((7514214926474921*cos(q4R))/36893488147419103232 + (4503599440548691*sin(q4R))/4503599627370496)*((9007199067919185*sin(q3R)*((23235800371559029388956996013805*cos(q1R))/40564819207303340847894502572032 - (17274190877287359225804725738355*sin(q1R))/162259276829213363391578010288128))/9007199254740992 + cos(q3R)*(cos(q2R)*((1917820484151683*cos(q1R))/18014398509481984 + (2579692110316253*sin(q1R))/4503599627370496) - (7514214926474921*sin(q2R)*((2579692110316253*cos(q1R))/4503599627370496 - (1917820484151683*sin(q1R))/18014398509481984))/36893488147419103232) + (7514214926474921*sin(q3R)*((7514214926474921*cos(q2R)*((2579692110316253*cos(q1R))/4503599627370496 - (1917820484151683*sin(q1R))/18014398509481984))/36893488147419103232 + sin(q2R)*((1917820484151683*cos(q1R))/18014398509481984 + (2579692110316253*sin(q1R))/4503599627370496)))/36893488147419103232)) - (7514214926474921*sin(q5R)*((7514214926474921*cos(q4R)*((9007199067919185*cos(q3R)*((23235800371559029388956996013805*cos(q1R))/40564819207303340847894502572032 - (17274190877287359225804725738355*sin(q1R))/162259276829213363391578010288128))/9007199254740992 + (7514214926474921*cos(q3R)*((7514214926474921*cos(q2R)*((2579692110316253*cos(q1R))/4503599627370496 - (1917820484151683*sin(q1R))/18014398509481984))/36893488147419103232 + sin(q2R)*((1917820484151683*cos(q1R))/18014398509481984 + (2579692110316253*sin(q1R))/4503599627370496)))/36893488147419103232 - sin(q3R)*(cos(q2R)*((1917820484151683*cos(q1R))/18014398509481984 + (2579692110316253*sin(q1R))/4503599627370496) - (7514214926474921*sin(q2R)*((2579692110316253*cos(q1R))/4503599627370496 - (1917820484151683*sin(q1R))/18014398509481984))/36893488147419103232)))/36893488147419103232 - ((234819211581865*cos(q4R))/1152921504606846976 + (9007199067919185*sin(q4R))/9007199254740992)*((129801982932889585091297864435361917839115294955*sin(q1R))/5986310706507378352962293074805895248510699696029696 - (174598797980560374072834504815488878557302284405*cos(q1R))/1496577676626844588240573268701473812127674924007424 + (67682029681889335677290557259385*cos(q2R)*((2579692110316253*cos(q1R))/4503599627370496 - (1917820484151683*sin(q1R))/18014398509481984))/332306998946228968225951765070086144 + (9007199067919185*sin(q2R)*((1917820484151683*cos(q1R))/18014398509481984 + (2579692110316253*sin(q1R))/4503599627370496))/9007199254740992) + ((4503599440548691*cos(q4R))/4503599627370496 - (7514214926474921*sin(q4R))/36893488147419103232)*((9007199067919185*sin(q3R)*((23235800371559029388956996013805*cos(q1R))/40564819207303340847894502572032 - (17274190877287359225804725738355*sin(q1R))/162259276829213363391578010288128))/9007199254740992 + cos(q3R)*(cos(q2R)*((1917820484151683*cos(q1R))/18014398509481984 + (2579692110316253*sin(q1R))/4503599627370496) - (7514214926474921*sin(q2R)*((2579692110316253*cos(q1R))/4503599627370496 - (1917820484151683*sin(q1R))/18014398509481984))/36893488147419103232) + (7514214926474921*sin(q3R)*((7514214926474921*cos(q2R)*((2579692110316253*cos(q1R))/4503599627370496 - (1917820484151683*sin(q1R))/18014398509481984))/36893488147419103232 + sin(q2R)*((1917820484151683*cos(q1R))/18014398509481984 + (2579692110316253*sin(q1R))/4503599627370496)))/36893488147419103232)))/36893488147419103232 + (9007199067919185*sin(q5R)*((273626851807209941619219010639387076236787289365779842797695875*cos(q1R))/56539106072908298546665520023773392506479484700019806659891398441363832832 - (203422408166946418981152780445187297537016008229516441756292125*sin(q1R))/226156424291633194186662080095093570025917938800079226639565593765455331328 - (81129635049124235038645691064225*cos(q3R)*((23235800371559029388956996013805*cos(q1R))/40564819207303340847894502572032 - (17274190877287359225804725738355*sin(q1R))/162259276829213363391578010288128))/81129638414606681695789005144064 + (2115063383689692319117831580025*sin(q3R)*((23235800371559029388956996013805*cos(q1R))/40564819207303340847894502572032 - (17274190877287359225804725738355*sin(q1R))/162259276829213363391578010288128))/10384593717069655257060992658440192 + (234819211581865*cos(q3R)*(cos(q2R)*((1917820484151683*cos(q1R))/18014398509481984 + (2579692110316253*sin(q1R))/4503599627370496) - (7514214926474921*sin(q2R)*((2579692110316253*cos(q1R))/4503599627370496 - (1917820484151683*sin(q1R))/18014398509481984))/36893488147419103232))/1152921504606846976 - (67682029681889335677290557259385*cos(q3R)*((7514214926474921*cos(q2R)*((2579692110316253*cos(q1R))/4503599627370496 - (1917820484151683*sin(q1R))/18014398509481984))/36893488147419103232 + sin(q2R)*((1917820484151683*cos(q1R))/18014398509481984 + (2579692110316253*sin(q1R))/4503599627370496)))/332306998946228968225951765070086144 + (9007199067919185*sin(q3R)*(cos(q2R)*((1917820484151683*cos(q1R))/18014398509481984 + (2579692110316253*sin(q1R))/4503599627370496) - (7514214926474921*sin(q2R)*((2579692110316253*cos(q1R))/4503599627370496 - (1917820484151683*sin(q1R))/18014398509481984))/36893488147419103232))/9007199254740992 + (1764482024691522628700660907665*sin(q3R)*((7514214926474921*cos(q2R)*((2579692110316253*cos(q1R))/4503599627370496 - (1917820484151683*sin(q1R))/18014398509481984))/36893488147419103232 + sin(q2R)*((1917820484151683*cos(q1R))/18014398509481984 + (2579692110316253*sin(q1R))/4503599627370496)))/42535295865117307932921825928971026432 - (106069577339469832923929692356850887620017617375*cos(q2R)*((2579692110316253*cos(q1R))/4503599627370496 - (1917820484151683*sin(q1R))/18014398509481984))/12554203470773361527671578846415332832204710888928069025792 - (14115856197532180673579726082375*sin(q2R)*((1917820484151683*cos(q1R))/18014398509481984 + (2579692110316253*sin(q1R))/4503599627370496))/340282366920938463463374607431768211456))/9007199254740992))/9007199254740992000 - (109198173955282063961996941994332957526645881091499469714283881779231664456243735535448036415347*sin(q3R)*((23235800371559029388956996013805*cos(q1R))/40564819207303340847894502572032 - (17274190877287359225804725738355*sin(q1R))/162259276829213363391578010288128))/2607406049708142190423610481164004046145879543892398400814259775173608063697070983914748641280000 - (81222263116692158804177042061221826384594597321566869716687*((4503599440548691*cos(q4R))/4503599627370496 - (7514214926474921*sin(q4R))/36893488147419103232)*((9007199067919185*sin(q3R)*((23235800371559029388956996013805*cos(q1R))/40564819207303340847894502572032 - (17274190877287359225804725738355*sin(q1R))/162259276829213363391578010288128))/9007199254740992 + cos(q3R)*(cos(q2R)*((1917820484151683*cos(q1R))/18014398509481984 + (2579692110316253*sin(q1R))/4503599627370496) - (7514214926474921*sin(q2R)*((2579692110316253*cos(q1R))/4503599627370496 - (1917820484151683*sin(q1R))/18014398509481984))/36893488147419103232) + (7514214926474921*sin(q3R)*((7514214926474921*cos(q2R)*((2579692110316253*cos(q1R))/4503599627370496 - (1917820484151683*sin(q1R))/18014398509481984))/36893488147419103232 + sin(q2R)*((1917820484151683*cos(q1R))/18014398509481984 + (2579692110316253*sin(q1R))/4503599627370496)))/36893488147419103232))/306499108173177771671669405430061836723747824436720435200000 - (81*((7514214926474921*cos(q4R))/36893488147419103232 + (4503599440548691*sin(q4R))/4503599627370496)*((9007199067919185*sin(q3R)*((23235800371559029388956996013805*cos(q1R))/40564819207303340847894502572032 - (17274190877287359225804725738355*sin(q1R))/162259276829213363391578010288128))/9007199254740992 + cos(q3R)*(cos(q2R)*((1917820484151683*cos(q1R))/18014398509481984 + (2579692110316253*sin(q1R))/4503599627370496) - (7514214926474921*sin(q2R)*((2579692110316253*cos(q1R))/4503599627370496 - (1917820484151683*sin(q1R))/18014398509481984))/36893488147419103232) + (7514214926474921*sin(q3R)*((7514214926474921*cos(q2R)*((2579692110316253*cos(q1R))/4503599627370496 - (1917820484151683*sin(q1R))/18014398509481984))/36893488147419103232 + sin(q2R)*((1917820484151683*cos(q1R))/18014398509481984 + (2579692110316253*sin(q1R))/4503599627370496)))/36893488147419103232))/2000 - (60617164743372705924380750591060836759586313939367162716784907429017787816377231*cos(q3R)*(cos(q2R)*((1917820484151683*cos(q1R))/18014398509481984 + (2579692110316253*sin(q1R))/4503599627370496) - (7514214926474921*sin(q2R)*((2579692110316253*cos(q1R))/4503599627370496 - (1917820484151683*sin(q1R))/18014398509481984))/36893488147419103232))/1447401115466452442794637312608598848165874808320507050493219800098914120499200000 + (347469655025336708709976918716104493695816557877713443586884917071777956519687017125887603*cos(q3R)*((7514214926474921*cos(q2R)*((2579692110316253*cos(q1R))/4503599627370496 - (1917820484151683*sin(q1R))/18014398509481984))/36893488147419103232 + sin(q2R)*((1917820484151683*cos(q1R))/18014398509481984 + (2579692110316253*sin(q1R))/4503599627370496)))/83436993590660550093555535397248129476668145404556748826056312805555458038306271485271956520960000 - (46241644459901303158631016767207157814229090534989303509431886332469146043*sin(q3R)*(cos(q2R)*((1917820484151683*cos(q1R))/18014398509481984 + (2579692110316253*sin(q1R))/4503599627370496) - (7514214926474921*sin(q2R)*((2579692110316253*cos(q1R))/4503599627370496 - (1917820484151683*sin(q1R))/18014398509481984))/36893488147419103232))/2261564242916331941866620800950935700259179388000792266395655937654553313280000 - (455490404115240510935077772268745492204390157443214084883134054419271951750419293234291596923751*sin(q3R)*((7514214926474921*cos(q2R)*((2579692110316253*cos(q1R))/4503599627370496 - (1917820484151683*sin(q1R))/18014398509481984))/36893488147419103232 + sin(q2R)*((1917820484151683*cos(q1R))/18014398509481984 + (2579692110316253*sin(q1R))/4503599627370496)))/53399675898022752059875542654238802865067613058916319248676040195555493144516013750574052173414400000 - (807520961047489018778067709720399904923771262077295170375712179706208528987338271217011451790113918662491539890779991*cos(q2R)*((2579692110316253*cos(q1R))/4503599627370496 - (1917820484151683*sin(q1R))/18014398509481984))/15760802478557791684911616040057445522031895708186178667179317361698288708598884244565706501953966256322651196122726400000 - (3*cos(q2R)*((1917820484151683*cos(q1R))/18014398509481984 + (2579692110316253*sin(q1R))/4503599627370496))/100 + (22542644779424763*sin(q2R)*((2579692110316253*cos(q1R))/4503599627370496 - (1917820484151683*sin(q1R))/18014398509481984))/3689348814741910323200 - (107465779053290185796889472867275736954369330186921663479979246519176992895505610212310958309481948671*sin(q2R)*((1917820484151683*cos(q1R))/18014398509481984 + (2579692110316253*sin(q1R))/4503599627370496))/427197407184182016479004341233910422920540904471330553989408321564443945156128110004592417387315200000 + (712008244765680093343103025701132101054572137019*cos(q5R)*((7514214926474921*cos(q4R)*((9007199067919185*cos(q3R)*((23235800371559029388956996013805*cos(q1R))/40564819207303340847894502572032 - (17274190877287359225804725738355*sin(q1R))/162259276829213363391578010288128))/9007199254740992 + (7514214926474921*cos(q3R)*((7514214926474921*cos(q2R)*((2579692110316253*cos(q1R))/4503599627370496 - (1917820484151683*sin(q1R))/18014398509481984))/36893488147419103232 + sin(q2R)*((1917820484151683*cos(q1R))/18014398509481984 + (2579692110316253*sin(q1R))/4503599627370496)))/36893488147419103232 - sin(q3R)*(cos(q2R)*((1917820484151683*cos(q1R))/18014398509481984 + (2579692110316253*sin(q1R))/4503599627370496) - (7514214926474921*sin(q2R)*((2579692110316253*cos(q1R))/4503599627370496 - (1917820484151683*sin(q1R))/18014398509481984))/36893488147419103232)))/36893488147419103232 - ((234819211581865*cos(q4R))/1152921504606846976 + (9007199067919185*sin(q4R))/9007199254740992)*((129801982932889585091297864435361917839115294955*sin(q1R))/5986310706507378352962293074805895248510699696029696 - (174598797980560374072834504815488878557302284405*cos(q1R))/1496577676626844588240573268701473812127674924007424 + (67682029681889335677290557259385*cos(q2R)*((2579692110316253*cos(q1R))/4503599627370496 - (1917820484151683*sin(q1R))/18014398509481984))/332306998946228968225951765070086144 + (9007199067919185*sin(q2R)*((1917820484151683*cos(q1R))/18014398509481984 + (2579692110316253*sin(q1R))/4503599627370496))/9007199254740992) + ((4503599440548691*cos(q4R))/4503599627370496 - (7514214926474921*sin(q4R))/36893488147419103232)*((9007199067919185*sin(q3R)*((23235800371559029388956996013805*cos(q1R))/40564819207303340847894502572032 - (17274190877287359225804725738355*sin(q1R))/162259276829213363391578010288128))/9007199254740992 + cos(q3R)*(cos(q2R)*((1917820484151683*cos(q1R))/18014398509481984 + (2579692110316253*sin(q1R))/4503599627370496) - (7514214926474921*sin(q2R)*((2579692110316253*cos(q1R))/4503599627370496 - (1917820484151683*sin(q1R))/18014398509481984))/36893488147419103232) + (7514214926474921*sin(q3R)*((7514214926474921*cos(q2R)*((2579692110316253*cos(q1R))/4503599627370496 - (1917820484151683*sin(q1R))/18014398509481984))/36893488147419103232 + sin(q2R)*((1917820484151683*cos(q1R))/18014398509481984 + (2579692110316253*sin(q1R))/4503599627370496)))/36893488147419103232)))/2451992865385422173373355243440494693789982595493763481600,(712008244765680093343103025701132101054572137019*cos(q5R)*(((4503599440548691*cos(q4R))/4503599627370496 - (7514214926474921*sin(q4R))/36893488147419103232)*(cos(q3R)*((32968958366167862000829996477285*cos(q2R))/40564819207303340847894502572032 - (7514214926474921*cos(q2R)*((1917820484151683*cos(q1R))/18014398509481984 + (2579692110316253*sin(q1R))/4503599627370496))/36893488147419103232 + sin(q2R)*((2579692110316253*cos(q1R))/4503599627370496 - (1917820484151683*sin(q1R))/18014398509481984)) - (7514214926474921*sin(q3R)*(cos(q2R)*((2579692110316253*cos(q1R))/4503599627370496 - (1917820484151683*sin(q1R))/18014398509481984) - (32968958366167862000829996477285*sin(q2R))/40564819207303340847894502572032 + (7514214926474921*sin(q2R)*((1917820484151683*cos(q1R))/18014398509481984 + (2579692110316253*sin(q1R))/4503599627370496))/36893488147419103232))/36893488147419103232) + ((234819211581865*cos(q4R))/1152921504606846976 + (9007199067919185*sin(q4R))/9007199254740992)*((9007199067919185*cos(q2R)*((2579692110316253*cos(q1R))/4503599627370496 - (1917820484151683*sin(q1R))/18014398509481984))/9007199254740992 - (296957971066013582975066703729047659005068212725*sin(q2R))/365375409332725729550921208179070754913983135744 + (67682029681889335677290557259385*sin(q2R)*((1917820484151683*cos(q1R))/18014398509481984 + (2579692110316253*sin(q1R))/4503599627370496))/332306998946228968225951765070086144) - (7514214926474921*cos(q4R)*((7514214926474921*cos(q3R)*(cos(q2R)*((2579692110316253*cos(q1R))/4503599627370496 - (1917820484151683*sin(q1R))/18014398509481984) - (32968958366167862000829996477285*sin(q2R))/40564819207303340847894502572032 + (7514214926474921*sin(q2R)*((1917820484151683*cos(q1R))/18014398509481984 + (2579692110316253*sin(q1R))/4503599627370496))/36893488147419103232))/36893488147419103232 + sin(q3R)*((32968958366167862000829996477285*cos(q2R))/40564819207303340847894502572032 - (7514214926474921*cos(q2R)*((1917820484151683*cos(q1R))/18014398509481984 + (2579692110316253*sin(q1R))/4503599627370496))/36893488147419103232 + sin(q2R)*((2579692110316253*cos(q1R))/4503599627370496 - (1917820484151683*sin(q1R))/18014398509481984))))/36893488147419103232))/2451992865385422173373355243440494693789982595493763481600 - (708606959079143690309338635695211374537059626293380223101122867230772593380567869745271054038604035886333341357936783642045437487647*sin(q2R))/3465837117651018574473017730178854629295546344219770718963099475768276634757032028799968007630174472621739013701754464786217697280000 - (19781375019700717200497997886371*cos(q2R))/811296384146066816957890051440640 + (48638874966763599*sin(q5R)*((234819211581865*cos(q3R)*((32968958366167862000829996477285*cos(q2R))/40564819207303340847894502572032 - (7514214926474921*cos(q2R)*((1917820484151683*cos(q1R))/18014398509481984 + (2579692110316253*sin(q1R))/4503599627370496))/36893488147419103232 + sin(q2R)*((2579692110316253*cos(q1R))/4503599627370496 - (1917820484151683*sin(q1R))/18014398509481984)))/1152921504606846976 - (465385075279251052437186083221547446448384963368966483726351875*sin(q2R))/13803492693581127574869511724554050904902217944340773110325048447598592 + (67682029681889335677290557259385*cos(q3R)*(cos(q2R)*((2579692110316253*cos(q1R))/4503599627370496 - (1917820484151683*sin(q1R))/18014398509481984) - (32968958366167862000829996477285*sin(q2R))/40564819207303340847894502572032 + (7514214926474921*sin(q2R)*((1917820484151683*cos(q1R))/18014398509481984 + (2579692110316253*sin(q1R))/4503599627370496))/36893488147419103232))/332306998946228968225951765070086144 + (9007199067919185*sin(q3R)*((32968958366167862000829996477285*cos(q2R))/40564819207303340847894502572032 - (7514214926474921*cos(q2R)*((1917820484151683*cos(q1R))/18014398509481984 + (2579692110316253*sin(q1R))/4503599627370496))/36893488147419103232 + sin(q2R)*((2579692110316253*cos(q1R))/4503599627370496 - (1917820484151683*sin(q1R))/18014398509481984)))/9007199254740992 - (1764482024691522628700660907665*sin(q3R)*(cos(q2R)*((2579692110316253*cos(q1R))/4503599627370496 - (1917820484151683*sin(q1R))/18014398509481984) - (32968958366167862000829996477285*sin(q2R))/40564819207303340847894502572032 + (7514214926474921*sin(q2R)*((1917820484151683*cos(q1R))/18014398509481984 + (2579692110316253*sin(q1R))/4503599627370496))/36893488147419103232))/42535295865117307932921825928971026432 + (14115856197532180673579726082375*cos(q2R)*((2579692110316253*cos(q1R))/4503599627370496 - (1917820484151683*sin(q1R))/18014398509481984))/340282366920938463463374607431768211456 + (106069577339469832923929692356850887620017617375*sin(q2R)*((1917820484151683*cos(q1R))/18014398509481984 + (2579692110316253*sin(q1R))/4503599627370496))/12554203470773361527671578846415332832204710888928069025792))/1801439850948198400 - (202883803014822867*sin(q5R)*(((4503599440548691*cos(q4R))/4503599627370496 - (7514214926474921*sin(q4R))/36893488147419103232)*(cos(q3R)*((32968958366167862000829996477285*cos(q2R))/40564819207303340847894502572032 - (7514214926474921*cos(q2R)*((1917820484151683*cos(q1R))/18014398509481984 + (2579692110316253*sin(q1R))/4503599627370496))/36893488147419103232 + sin(q2R)*((2579692110316253*cos(q1R))/4503599627370496 - (1917820484151683*sin(q1R))/18014398509481984)) - (7514214926474921*sin(q3R)*(cos(q2R)*((2579692110316253*cos(q1R))/4503599627370496 - (1917820484151683*sin(q1R))/18014398509481984) - (32968958366167862000829996477285*sin(q2R))/40564819207303340847894502572032 + (7514214926474921*sin(q2R)*((1917820484151683*cos(q1R))/18014398509481984 + (2579692110316253*sin(q1R))/4503599627370496))/36893488147419103232))/36893488147419103232) + ((234819211581865*cos(q4R))/1152921504606846976 + (9007199067919185*sin(q4R))/9007199254740992)*((9007199067919185*cos(q2R)*((2579692110316253*cos(q1R))/4503599627370496 - (1917820484151683*sin(q1R))/18014398509481984))/9007199254740992 - (296957971066013582975066703729047659005068212725*sin(q2R))/365375409332725729550921208179070754913983135744 + (67682029681889335677290557259385*sin(q2R)*((1917820484151683*cos(q1R))/18014398509481984 + (2579692110316253*sin(q1R))/4503599627370496))/332306998946228968225951765070086144) - (7514214926474921*cos(q4R)*((7514214926474921*cos(q3R)*(cos(q2R)*((2579692110316253*cos(q1R))/4503599627370496 - (1917820484151683*sin(q1R))/18014398509481984) - (32968958366167862000829996477285*sin(q2R))/40564819207303340847894502572032 + (7514214926474921*sin(q2R)*((1917820484151683*cos(q1R))/18014398509481984 + (2579692110316253*sin(q1R))/4503599627370496))/36893488147419103232))/36893488147419103232 + sin(q3R)*((32968958366167862000829996477285*cos(q2R))/40564819207303340847894502572032 - (7514214926474921*cos(q2R)*((1917820484151683*cos(q1R))/18014398509481984 + (2579692110316253*sin(q1R))/4503599627370496))/36893488147419103232 + sin(q2R)*((2579692110316253*cos(q1R))/4503599627370496 - (1917820484151683*sin(q1R))/18014398509481984))))/36893488147419103232))/36893488147419103232000 - (27*cos(q5R)*(((9007199067919185*cos(q4R))/9007199254740992 - (234819211581865*sin(q4R))/1152921504606846976)*((9007199067919185*cos(q2R)*((2579692110316253*cos(q1R))/4503599627370496 - (1917820484151683*sin(q1R))/18014398509481984))/9007199254740992 - (296957971066013582975066703729047659005068212725*sin(q2R))/365375409332725729550921208179070754913983135744 + (67682029681889335677290557259385*sin(q2R)*((1917820484151683*cos(q1R))/18014398509481984 + (2579692110316253*sin(q1R))/4503599627370496))/332306998946228968225951765070086144) - ((7514214926474921*cos(q4R))/36893488147419103232 + (4503599440548691*sin(q4R))/4503599627370496)*(cos(q3R)*((32968958366167862000829996477285*cos(q2R))/40564819207303340847894502572032 - (7514214926474921*cos(q2R)*((1917820484151683*cos(q1R))/18014398509481984 + (2579692110316253*sin(q1R))/4503599627370496))/36893488147419103232 + sin(q2R)*((2579692110316253*cos(q1R))/4503599627370496 - (1917820484151683*sin(q1R))/18014398509481984)) - (7514214926474921*sin(q3R)*(cos(q2R)*((2579692110316253*cos(q1R))/4503599627370496 - (1917820484151683*sin(q1R))/18014398509481984) - (32968958366167862000829996477285*sin(q2R))/40564819207303340847894502572032 + (7514214926474921*sin(q2R)*((1917820484151683*cos(q1R))/18014398509481984 + (2579692110316253*sin(q1R))/4503599627370496))/36893488147419103232))/36893488147419103232) + (7514214926474921*sin(q4R)*((7514214926474921*cos(q3R)*(cos(q2R)*((2579692110316253*cos(q1R))/4503599627370496 - (1917820484151683*sin(q1R))/18014398509481984) - (32968958366167862000829996477285*sin(q2R))/40564819207303340847894502572032 + (7514214926474921*sin(q2R)*((1917820484151683*cos(q1R))/18014398509481984 + (2579692110316253*sin(q1R))/4503599627370496))/36893488147419103232))/36893488147419103232 + sin(q3R)*((32968958366167862000829996477285*cos(q2R))/40564819207303340847894502572032 - (7514214926474921*cos(q2R)*((1917820484151683*cos(q1R))/18014398509481984 + (2579692110316253*sin(q1R))/4503599627370496))/36893488147419103232 + sin(q2R)*((2579692110316253*cos(q1R))/4503599627370496 - (1917820484151683*sin(q1R))/18014398509481984))))/36893488147419103232))/1000 + (2436553109258773196144549622003023*cos(q6R)*(sin(q5R)*(((9007199067919185*cos(q4R))/9007199254740992 - (234819211581865*sin(q4R))/1152921504606846976)*((9007199067919185*cos(q2R)*((2579692110316253*cos(q1R))/4503599627370496 - (1917820484151683*sin(q1R))/18014398509481984))/9007199254740992 - (296957971066013582975066703729047659005068212725*sin(q2R))/365375409332725729550921208179070754913983135744 + (67682029681889335677290557259385*sin(q2R)*((1917820484151683*cos(q1R))/18014398509481984 + (2579692110316253*sin(q1R))/4503599627370496))/332306998946228968225951765070086144) - ((7514214926474921*cos(q4R))/36893488147419103232 + (4503599440548691*sin(q4R))/4503599627370496)*(cos(q3R)*((32968958366167862000829996477285*cos(q2R))/40564819207303340847894502572032 - (7514214926474921*cos(q2R)*((1917820484151683*cos(q1R))/18014398509481984 + (2579692110316253*sin(q1R))/4503599627370496))/36893488147419103232 + sin(q2R)*((2579692110316253*cos(q1R))/4503599627370496 - (1917820484151683*sin(q1R))/18014398509481984)) - (7514214926474921*sin(q3R)*(cos(q2R)*((2579692110316253*cos(q1R))/4503599627370496 - (1917820484151683*sin(q1R))/18014398509481984) - (32968958366167862000829996477285*sin(q2R))/40564819207303340847894502572032 + (7514214926474921*sin(q2R)*((1917820484151683*cos(q1R))/18014398509481984 + (2579692110316253*sin(q1R))/4503599627370496))/36893488147419103232))/36893488147419103232) + (7514214926474921*sin(q4R)*((7514214926474921*cos(q3R)*(cos(q2R)*((2579692110316253*cos(q1R))/4503599627370496 - (1917820484151683*sin(q1R))/18014398509481984) - (32968958366167862000829996477285*sin(q2R))/40564819207303340847894502572032 + (7514214926474921*sin(q2R)*((1917820484151683*cos(q1R))/18014398509481984 + (2579692110316253*sin(q1R))/4503599627370496))/36893488147419103232))/36893488147419103232 + sin(q3R)*((32968958366167862000829996477285*cos(q2R))/40564819207303340847894502572032 - (7514214926474921*cos(q2R)*((1917820484151683*cos(q1R))/18014398509481984 + (2579692110316253*sin(q1R))/4503599627370496))/36893488147419103232 + sin(q2R)*((2579692110316253*cos(q1R))/4503599627370496 - (1917820484151683*sin(q1R))/18014398509481984))))/36893488147419103232) - (7514214926474921*cos(q5R)*(((4503599440548691*cos(q4R))/4503599627370496 - (7514214926474921*sin(q4R))/36893488147419103232)*(cos(q3R)*((32968958366167862000829996477285*cos(q2R))/40564819207303340847894502572032 - (7514214926474921*cos(q2R)*((1917820484151683*cos(q1R))/18014398509481984 + (2579692110316253*sin(q1R))/4503599627370496))/36893488147419103232 + sin(q2R)*((2579692110316253*cos(q1R))/4503599627370496 - (1917820484151683*sin(q1R))/18014398509481984)) - (7514214926474921*sin(q3R)*(cos(q2R)*((2579692110316253*cos(q1R))/4503599627370496 - (1917820484151683*sin(q1R))/18014398509481984) - (32968958366167862000829996477285*sin(q2R))/40564819207303340847894502572032 + (7514214926474921*sin(q2R)*((1917820484151683*cos(q1R))/18014398509481984 + (2579692110316253*sin(q1R))/4503599627370496))/36893488147419103232))/36893488147419103232) + ((234819211581865*cos(q4R))/1152921504606846976 + (9007199067919185*sin(q4R))/9007199254740992)*((9007199067919185*cos(q2R)*((2579692110316253*cos(q1R))/4503599627370496 - (1917820484151683*sin(q1R))/18014398509481984))/9007199254740992 - (296957971066013582975066703729047659005068212725*sin(q2R))/365375409332725729550921208179070754913983135744 + (67682029681889335677290557259385*sin(q2R)*((1917820484151683*cos(q1R))/18014398509481984 + (2579692110316253*sin(q1R))/4503599627370496))/332306998946228968225951765070086144) - (7514214926474921*cos(q4R)*((7514214926474921*cos(q3R)*(cos(q2R)*((2579692110316253*cos(q1R))/4503599627370496 - (1917820484151683*sin(q1R))/18014398509481984) - (32968958366167862000829996477285*sin(q2R))/40564819207303340847894502572032 + (7514214926474921*sin(q2R)*((1917820484151683*cos(q1R))/18014398509481984 + (2579692110316253*sin(q1R))/4503599627370496))/36893488147419103232))/36893488147419103232 + sin(q3R)*((32968958366167862000829996477285*cos(q2R))/40564819207303340847894502572032 - (7514214926474921*cos(q2R)*((1917820484151683*cos(q1R))/18014398509481984 + (2579692110316253*sin(q1R))/4503599627370496))/36893488147419103232 + sin(q2R)*((2579692110316253*cos(q1R))/4503599627370496 - (1917820484151683*sin(q1R))/18014398509481984))))/36893488147419103232))/36893488147419103232 + (9007199067919185*cos(q5R)*((234819211581865*cos(q3R)*((32968958366167862000829996477285*cos(q2R))/40564819207303340847894502572032 - (7514214926474921*cos(q2R)*((1917820484151683*cos(q1R))/18014398509481984 + (2579692110316253*sin(q1R))/4503599627370496))/36893488147419103232 + sin(q2R)*((2579692110316253*cos(q1R))/4503599627370496 - (1917820484151683*sin(q1R))/18014398509481984)))/1152921504606846976 - (465385075279251052437186083221547446448384963368966483726351875*sin(q2R))/13803492693581127574869511724554050904902217944340773110325048447598592 + (67682029681889335677290557259385*cos(q3R)*(cos(q2R)*((2579692110316253*cos(q1R))/4503599627370496 - (1917820484151683*sin(q1R))/18014398509481984) - (32968958366167862000829996477285*sin(q2R))/40564819207303340847894502572032 + (7514214926474921*sin(q2R)*((1917820484151683*cos(q1R))/18014398509481984 + (2579692110316253*sin(q1R))/4503599627370496))/36893488147419103232))/332306998946228968225951765070086144 + (9007199067919185*sin(q3R)*((32968958366167862000829996477285*cos(q2R))/40564819207303340847894502572032 - (7514214926474921*cos(q2R)*((1917820484151683*cos(q1R))/18014398509481984 + (2579692110316253*sin(q1R))/4503599627370496))/36893488147419103232 + sin(q2R)*((2579692110316253*cos(q1R))/4503599627370496 - (1917820484151683*sin(q1R))/18014398509481984)))/9007199254740992 - (1764482024691522628700660907665*sin(q3R)*(cos(q2R)*((2579692110316253*cos(q1R))/4503599627370496 - (1917820484151683*sin(q1R))/18014398509481984) - (32968958366167862000829996477285*sin(q2R))/40564819207303340847894502572032 + (7514214926474921*sin(q2R)*((1917820484151683*cos(q1R))/18014398509481984 + (2579692110316253*sin(q1R))/4503599627370496))/36893488147419103232))/42535295865117307932921825928971026432 + (14115856197532180673579726082375*cos(q2R)*((2579692110316253*cos(q1R))/4503599627370496 - (1917820484151683*sin(q1R))/18014398509481984))/340282366920938463463374607431768211456 + (106069577339469832923929692356850887620017617375*sin(q2R)*((1917820484151683*cos(q1R))/18014398509481984 + (2579692110316253*sin(q1R))/4503599627370496))/12554203470773361527671578846415332832204710888928069025792))/9007199254740992))/332306998946228968225951765070086144000 - (81222263116692158804177042061221826384594597321566869716687*((4503599440548691*cos(q4R))/4503599627370496 - (7514214926474921*sin(q4R))/36893488147419103232)*(cos(q3R)*((32968958366167862000829996477285*cos(q2R))/40564819207303340847894502572032 - (7514214926474921*cos(q2R)*((1917820484151683*cos(q1R))/18014398509481984 + (2579692110316253*sin(q1R))/4503599627370496))/36893488147419103232 + sin(q2R)*((2579692110316253*cos(q1R))/4503599627370496 - (1917820484151683*sin(q1R))/18014398509481984)) - (7514214926474921*sin(q3R)*(cos(q2R)*((2579692110316253*cos(q1R))/4503599627370496 - (1917820484151683*sin(q1R))/18014398509481984) - (32968958366167862000829996477285*sin(q2R))/40564819207303340847894502572032 + (7514214926474921*sin(q2R)*((1917820484151683*cos(q1R))/18014398509481984 + (2579692110316253*sin(q1R))/4503599627370496))/36893488147419103232))/36893488147419103232))/306499108173177771671669405430061836723747824436720435200000 - (81*((7514214926474921*cos(q4R))/36893488147419103232 + (4503599440548691*sin(q4R))/4503599627370496)*(cos(q3R)*((32968958366167862000829996477285*cos(q2R))/40564819207303340847894502572032 - (7514214926474921*cos(q2R)*((1917820484151683*cos(q1R))/18014398509481984 + (2579692110316253*sin(q1R))/4503599627370496))/36893488147419103232 + sin(q2R)*((2579692110316253*cos(q1R))/4503599627370496 - (1917820484151683*sin(q1R))/18014398509481984)) - (7514214926474921*sin(q3R)*(cos(q2R)*((2579692110316253*cos(q1R))/4503599627370496 - (1917820484151683*sin(q1R))/18014398509481984) - (32968958366167862000829996477285*sin(q2R))/40564819207303340847894502572032 + (7514214926474921*sin(q2R)*((1917820484151683*cos(q1R))/18014398509481984 + (2579692110316253*sin(q1R))/4503599627370496))/36893488147419103232))/36893488147419103232))/2000 - (94754841554645069948206780163139*sin(q5R)*(((9007199067919185*cos(q4R))/9007199254740992 - (234819211581865*sin(q4R))/1152921504606846976)*((9007199067919185*cos(q2R)*((2579692110316253*cos(q1R))/4503599627370496 - (1917820484151683*sin(q1R))/18014398509481984))/9007199254740992 - (296957971066013582975066703729047659005068212725*sin(q2R))/365375409332725729550921208179070754913983135744 + (67682029681889335677290557259385*sin(q2R)*((1917820484151683*cos(q1R))/18014398509481984 + (2579692110316253*sin(q1R))/4503599627370496))/332306998946228968225951765070086144) - ((7514214926474921*cos(q4R))/36893488147419103232 + (4503599440548691*sin(q4R))/4503599627370496)*(cos(q3R)*((32968958366167862000829996477285*cos(q2R))/40564819207303340847894502572032 - (7514214926474921*cos(q2R)*((1917820484151683*cos(q1R))/18014398509481984 + (2579692110316253*sin(q1R))/4503599627370496))/36893488147419103232 + sin(q2R)*((2579692110316253*cos(q1R))/4503599627370496 - (1917820484151683*sin(q1R))/18014398509481984)) - (7514214926474921*sin(q3R)*(cos(q2R)*((2579692110316253*cos(q1R))/4503599627370496 - (1917820484151683*sin(q1R))/18014398509481984) - (32968958366167862000829996477285*sin(q2R))/40564819207303340847894502572032 + (7514214926474921*sin(q2R)*((1917820484151683*cos(q1R))/18014398509481984 + (2579692110316253*sin(q1R))/4503599627370496))/36893488147419103232))/36893488147419103232) + (7514214926474921*sin(q4R)*((7514214926474921*cos(q3R)*(cos(q2R)*((2579692110316253*cos(q1R))/4503599627370496 - (1917820484151683*sin(q1R))/18014398509481984) - (32968958366167862000829996477285*sin(q2R))/40564819207303340847894502572032 + (7514214926474921*sin(q2R)*((1917820484151683*cos(q1R))/18014398509481984 + (2579692110316253*sin(q1R))/4503599627370496))/36893488147419103232))/36893488147419103232 + sin(q3R)*((32968958366167862000829996477285*cos(q2R))/40564819207303340847894502572032 - (7514214926474921*cos(q2R)*((1917820484151683*cos(q1R))/18014398509481984 + (2579692110316253*sin(q1R))/4503599627370496))/36893488147419103232 + sin(q2R)*((2579692110316253*cos(q1R))/4503599627370496 - (1917820484151683*sin(q1R))/18014398509481984))))/36893488147419103232))/66461399789245793645190353014017228800 + (81*((9007199067919185*cos(q4R))/9007199254740992 - (234819211581865*sin(q4R))/1152921504606846976)*((9007199067919185*cos(q2R)*((2579692110316253*cos(q1R))/4503599627370496 - (1917820484151683*sin(q1R))/18014398509481984))/9007199254740992 - (296957971066013582975066703729047659005068212725*sin(q2R))/365375409332725729550921208179070754913983135744 + (67682029681889335677290557259385*sin(q2R)*((1917820484151683*cos(q1R))/18014398509481984 + (2579692110316253*sin(q1R))/4503599627370496))/332306998946228968225951765070086144))/2000 - (81222263116692158804177042061221826384594597321566869716687*((234819211581865*cos(q4R))/1152921504606846976 + (9007199067919185*sin(q4R))/9007199254740992)*((9007199067919185*cos(q2R)*((2579692110316253*cos(q1R))/4503599627370496 - (1917820484151683*sin(q1R))/18014398509481984))/9007199254740992 - (296957971066013582975066703729047659005068212725*sin(q2R))/365375409332725729550921208179070754913983135744 + (67682029681889335677290557259385*sin(q2R)*((1917820484151683*cos(q1R))/18014398509481984 + (2579692110316253*sin(q1R))/4503599627370496))/332306998946228968225951765070086144))/306499108173177771671669405430061836723747824436720435200000 + (27*cos(q6R)*((7514214926474921*sin(q5R)*(((4503599440548691*cos(q4R))/4503599627370496 - (7514214926474921*sin(q4R))/36893488147419103232)*(cos(q3R)*((32968958366167862000829996477285*cos(q2R))/40564819207303340847894502572032 - (7514214926474921*cos(q2R)*((1917820484151683*cos(q1R))/18014398509481984 + (2579692110316253*sin(q1R))/4503599627370496))/36893488147419103232 + sin(q2R)*((2579692110316253*cos(q1R))/4503599627370496 - (1917820484151683*sin(q1R))/18014398509481984)) - (7514214926474921*sin(q3R)*(cos(q2R)*((2579692110316253*cos(q1R))/4503599627370496 - (1917820484151683*sin(q1R))/18014398509481984) - (32968958366167862000829996477285*sin(q2R))/40564819207303340847894502572032 + (7514214926474921*sin(q2R)*((1917820484151683*cos(q1R))/18014398509481984 + (2579692110316253*sin(q1R))/4503599627370496))/36893488147419103232))/36893488147419103232) + ((234819211581865*cos(q4R))/1152921504606846976 + (9007199067919185*sin(q4R))/9007199254740992)*((9007199067919185*cos(q2R)*((2579692110316253*cos(q1R))/4503599627370496 - (1917820484151683*sin(q1R))/18014398509481984))/9007199254740992 - (296957971066013582975066703729047659005068212725*sin(q2R))/365375409332725729550921208179070754913983135744 + (67682029681889335677290557259385*sin(q2R)*((1917820484151683*cos(q1R))/18014398509481984 + (2579692110316253*sin(q1R))/4503599627370496))/332306998946228968225951765070086144) - (7514214926474921*cos(q4R)*((7514214926474921*cos(q3R)*(cos(q2R)*((2579692110316253*cos(q1R))/4503599627370496 - (1917820484151683*sin(q1R))/18014398509481984) - (32968958366167862000829996477285*sin(q2R))/40564819207303340847894502572032 + (7514214926474921*sin(q2R)*((1917820484151683*cos(q1R))/18014398509481984 + (2579692110316253*sin(q1R))/4503599627370496))/36893488147419103232))/36893488147419103232 + sin(q3R)*((32968958366167862000829996477285*cos(q2R))/40564819207303340847894502572032 - (7514214926474921*cos(q2R)*((1917820484151683*cos(q1R))/18014398509481984 + (2579692110316253*sin(q1R))/4503599627370496))/36893488147419103232 + sin(q2R)*((2579692110316253*cos(q1R))/4503599627370496 - (1917820484151683*sin(q1R))/18014398509481984))))/36893488147419103232))/36893488147419103232 - (9007199067919185*sin(q5R)*((234819211581865*cos(q3R)*((32968958366167862000829996477285*cos(q2R))/40564819207303340847894502572032 - (7514214926474921*cos(q2R)*((1917820484151683*cos(q1R))/18014398509481984 + (2579692110316253*sin(q1R))/4503599627370496))/36893488147419103232 + sin(q2R)*((2579692110316253*cos(q1R))/4503599627370496 - (1917820484151683*sin(q1R))/18014398509481984)))/1152921504606846976 - (465385075279251052437186083221547446448384963368966483726351875*sin(q2R))/13803492693581127574869511724554050904902217944340773110325048447598592 + (67682029681889335677290557259385*cos(q3R)*(cos(q2R)*((2579692110316253*cos(q1R))/4503599627370496 - (1917820484151683*sin(q1R))/18014398509481984) - (32968958366167862000829996477285*sin(q2R))/40564819207303340847894502572032 + (7514214926474921*sin(q2R)*((1917820484151683*cos(q1R))/18014398509481984 + (2579692110316253*sin(q1R))/4503599627370496))/36893488147419103232))/332306998946228968225951765070086144 + (9007199067919185*sin(q3R)*((32968958366167862000829996477285*cos(q2R))/40564819207303340847894502572032 - (7514214926474921*cos(q2R)*((1917820484151683*cos(q1R))/18014398509481984 + (2579692110316253*sin(q1R))/4503599627370496))/36893488147419103232 + sin(q2R)*((2579692110316253*cos(q1R))/4503599627370496 - (1917820484151683*sin(q1R))/18014398509481984)))/9007199254740992 - (1764482024691522628700660907665*sin(q3R)*(cos(q2R)*((2579692110316253*cos(q1R))/4503599627370496 - (1917820484151683*sin(q1R))/18014398509481984) - (32968958366167862000829996477285*sin(q2R))/40564819207303340847894502572032 + (7514214926474921*sin(q2R)*((1917820484151683*cos(q1R))/18014398509481984 + (2579692110316253*sin(q1R))/4503599627370496))/36893488147419103232))/42535295865117307932921825928971026432 + (14115856197532180673579726082375*cos(q2R)*((2579692110316253*cos(q1R))/4503599627370496 - (1917820484151683*sin(q1R))/18014398509481984))/340282366920938463463374607431768211456 + (106069577339469832923929692356850887620017617375*sin(q2R)*((1917820484151683*cos(q1R))/18014398509481984 + (2579692110316253*sin(q1R))/4503599627370496))/12554203470773361527671578846415332832204710888928069025792))/9007199254740992 + cos(q5R)*(((9007199067919185*cos(q4R))/9007199254740992 - (234819211581865*sin(q4R))/1152921504606846976)*((9007199067919185*cos(q2R)*((2579692110316253*cos(q1R))/4503599627370496 - (1917820484151683*sin(q1R))/18014398509481984))/9007199254740992 - (296957971066013582975066703729047659005068212725*sin(q2R))/365375409332725729550921208179070754913983135744 + (67682029681889335677290557259385*sin(q2R)*((1917820484151683*cos(q1R))/18014398509481984 + (2579692110316253*sin(q1R))/4503599627370496))/332306998946228968225951765070086144) - ((7514214926474921*cos(q4R))/36893488147419103232 + (4503599440548691*sin(q4R))/4503599627370496)*(cos(q3R)*((32968958366167862000829996477285*cos(q2R))/40564819207303340847894502572032 - (7514214926474921*cos(q2R)*((1917820484151683*cos(q1R))/18014398509481984 + (2579692110316253*sin(q1R))/4503599627370496))/36893488147419103232 + sin(q2R)*((2579692110316253*cos(q1R))/4503599627370496 - (1917820484151683*sin(q1R))/18014398509481984)) - (7514214926474921*sin(q3R)*(cos(q2R)*((2579692110316253*cos(q1R))/4503599627370496 - (1917820484151683*sin(q1R))/18014398509481984) - (32968958366167862000829996477285*sin(q2R))/40564819207303340847894502572032 + (7514214926474921*sin(q2R)*((1917820484151683*cos(q1R))/18014398509481984 + (2579692110316253*sin(q1R))/4503599627370496))/36893488147419103232))/36893488147419103232) + (7514214926474921*sin(q4R)*((7514214926474921*cos(q3R)*(cos(q2R)*((2579692110316253*cos(q1R))/4503599627370496 - (1917820484151683*sin(q1R))/18014398509481984) - (32968958366167862000829996477285*sin(q2R))/40564819207303340847894502572032 + (7514214926474921*sin(q2R)*((1917820484151683*cos(q1R))/18014398509481984 + (2579692110316253*sin(q1R))/4503599627370496))/36893488147419103232))/36893488147419103232 + sin(q3R)*((32968958366167862000829996477285*cos(q2R))/40564819207303340847894502572032 - (7514214926474921*cos(q2R)*((1917820484151683*cos(q1R))/18014398509481984 + (2579692110316253*sin(q1R))/4503599627370496))/36893488147419103232 + sin(q2R)*((2579692110316253*cos(q1R))/4503599627370496 - (1917820484151683*sin(q1R))/18014398509481984))))/36893488147419103232)))/1000 + (202883803014822867*sin(q6R)*(sin(q5R)*(((9007199067919185*cos(q4R))/9007199254740992 - (234819211581865*sin(q4R))/1152921504606846976)*((9007199067919185*cos(q2R)*((2579692110316253*cos(q1R))/4503599627370496 - (1917820484151683*sin(q1R))/18014398509481984))/9007199254740992 - (296957971066013582975066703729047659005068212725*sin(q2R))/365375409332725729550921208179070754913983135744 + (67682029681889335677290557259385*sin(q2R)*((1917820484151683*cos(q1R))/18014398509481984 + (2579692110316253*sin(q1R))/4503599627370496))/332306998946228968225951765070086144) - ((7514214926474921*cos(q4R))/36893488147419103232 + (4503599440548691*sin(q4R))/4503599627370496)*(cos(q3R)*((32968958366167862000829996477285*cos(q2R))/40564819207303340847894502572032 - (7514214926474921*cos(q2R)*((1917820484151683*cos(q1R))/18014398509481984 + (2579692110316253*sin(q1R))/4503599627370496))/36893488147419103232 + sin(q2R)*((2579692110316253*cos(q1R))/4503599627370496 - (1917820484151683*sin(q1R))/18014398509481984)) - (7514214926474921*sin(q3R)*(cos(q2R)*((2579692110316253*cos(q1R))/4503599627370496 - (1917820484151683*sin(q1R))/18014398509481984) - (32968958366167862000829996477285*sin(q2R))/40564819207303340847894502572032 + (7514214926474921*sin(q2R)*((1917820484151683*cos(q1R))/18014398509481984 + (2579692110316253*sin(q1R))/4503599627370496))/36893488147419103232))/36893488147419103232) + (7514214926474921*sin(q4R)*((7514214926474921*cos(q3R)*(cos(q2R)*((2579692110316253*cos(q1R))/4503599627370496 - (1917820484151683*sin(q1R))/18014398509481984) - (32968958366167862000829996477285*sin(q2R))/40564819207303340847894502572032 + (7514214926474921*sin(q2R)*((1917820484151683*cos(q1R))/18014398509481984 + (2579692110316253*sin(q1R))/4503599627370496))/36893488147419103232))/36893488147419103232 + sin(q3R)*((32968958366167862000829996477285*cos(q2R))/40564819207303340847894502572032 - (7514214926474921*cos(q2R)*((1917820484151683*cos(q1R))/18014398509481984 + (2579692110316253*sin(q1R))/4503599627370496))/36893488147419103232 + sin(q2R)*((2579692110316253*cos(q1R))/4503599627370496 - (1917820484151683*sin(q1R))/18014398509481984))))/36893488147419103232) - (7514214926474921*cos(q5R)*(((4503599440548691*cos(q4R))/4503599627370496 - (7514214926474921*sin(q4R))/36893488147419103232)*(cos(q3R)*((32968958366167862000829996477285*cos(q2R))/40564819207303340847894502572032 - (7514214926474921*cos(q2R)*((1917820484151683*cos(q1R))/18014398509481984 + (2579692110316253*sin(q1R))/4503599627370496))/36893488147419103232 + sin(q2R)*((2579692110316253*cos(q1R))/4503599627370496 - (1917820484151683*sin(q1R))/18014398509481984)) - (7514214926474921*sin(q3R)*(cos(q2R)*((2579692110316253*cos(q1R))/4503599627370496 - (1917820484151683*sin(q1R))/18014398509481984) - (32968958366167862000829996477285*sin(q2R))/40564819207303340847894502572032 + (7514214926474921*sin(q2R)*((1917820484151683*cos(q1R))/18014398509481984 + (2579692110316253*sin(q1R))/4503599627370496))/36893488147419103232))/36893488147419103232) + ((234819211581865*cos(q4R))/1152921504606846976 + (9007199067919185*sin(q4R))/9007199254740992)*((9007199067919185*cos(q2R)*((2579692110316253*cos(q1R))/4503599627370496 - (1917820484151683*sin(q1R))/18014398509481984))/9007199254740992 - (296957971066013582975066703729047659005068212725*sin(q2R))/365375409332725729550921208179070754913983135744 + (67682029681889335677290557259385*sin(q2R)*((1917820484151683*cos(q1R))/18014398509481984 + (2579692110316253*sin(q1R))/4503599627370496))/332306998946228968225951765070086144) - (7514214926474921*cos(q4R)*((7514214926474921*cos(q3R)*(cos(q2R)*((2579692110316253*cos(q1R))/4503599627370496 - (1917820484151683*sin(q1R))/18014398509481984) - (32968958366167862000829996477285*sin(q2R))/40564819207303340847894502572032 + (7514214926474921*sin(q2R)*((1917820484151683*cos(q1R))/18014398509481984 + (2579692110316253*sin(q1R))/4503599627370496))/36893488147419103232))/36893488147419103232 + sin(q3R)*((32968958366167862000829996477285*cos(q2R))/40564819207303340847894502572032 - (7514214926474921*cos(q2R)*((1917820484151683*cos(q1R))/18014398509481984 + (2579692110316253*sin(q1R))/4503599627370496))/36893488147419103232 + sin(q2R)*((2579692110316253*cos(q1R))/4503599627370496 - (1917820484151683*sin(q1R))/18014398509481984))))/36893488147419103232))/36893488147419103232 + (9007199067919185*cos(q5R)*((234819211581865*cos(q3R)*((32968958366167862000829996477285*cos(q2R))/40564819207303340847894502572032 - (7514214926474921*cos(q2R)*((1917820484151683*cos(q1R))/18014398509481984 + (2579692110316253*sin(q1R))/4503599627370496))/36893488147419103232 + sin(q2R)*((2579692110316253*cos(q1R))/4503599627370496 - (1917820484151683*sin(q1R))/18014398509481984)))/1152921504606846976 - (465385075279251052437186083221547446448384963368966483726351875*sin(q2R))/13803492693581127574869511724554050904902217944340773110325048447598592 + (67682029681889335677290557259385*cos(q3R)*(cos(q2R)*((2579692110316253*cos(q1R))/4503599627370496 - (1917820484151683*sin(q1R))/18014398509481984) - (32968958366167862000829996477285*sin(q2R))/40564819207303340847894502572032 + (7514214926474921*sin(q2R)*((1917820484151683*cos(q1R))/18014398509481984 + (2579692110316253*sin(q1R))/4503599627370496))/36893488147419103232))/332306998946228968225951765070086144 + (9007199067919185*sin(q3R)*((32968958366167862000829996477285*cos(q2R))/40564819207303340847894502572032 - (7514214926474921*cos(q2R)*((1917820484151683*cos(q1R))/18014398509481984 + (2579692110316253*sin(q1R))/4503599627370496))/36893488147419103232 + sin(q2R)*((2579692110316253*cos(q1R))/4503599627370496 - (1917820484151683*sin(q1R))/18014398509481984)))/9007199254740992 - (1764482024691522628700660907665*sin(q3R)*(cos(q2R)*((2579692110316253*cos(q1R))/4503599627370496 - (1917820484151683*sin(q1R))/18014398509481984) - (32968958366167862000829996477285*sin(q2R))/40564819207303340847894502572032 + (7514214926474921*sin(q2R)*((1917820484151683*cos(q1R))/18014398509481984 + (2579692110316253*sin(q1R))/4503599627370496))/36893488147419103232))/42535295865117307932921825928971026432 + (14115856197532180673579726082375*cos(q2R)*((2579692110316253*cos(q1R))/4503599627370496 - (1917820484151683*sin(q1R))/18014398509481984))/340282366920938463463374607431768211456 + (106069577339469832923929692356850887620017617375*sin(q2R)*((1917820484151683*cos(q1R))/18014398509481984 + (2579692110316253*sin(q1R))/4503599627370496))/12554203470773361527671578846415332832204710888928069025792))/9007199254740992))/36893488147419103232000 - (584133382113593486367040631332731*cos(q6R)*((9007199067919185*((4503599440548691*cos(q4R))/4503599627370496 - (7514214926474921*sin(q4R))/36893488147419103232)*(cos(q3R)*((32968958366167862000829996477285*cos(q2R))/40564819207303340847894502572032 - (7514214926474921*cos(q2R)*((1917820484151683*cos(q1R))/18014398509481984 + (2579692110316253*sin(q1R))/4503599627370496))/36893488147419103232 + sin(q2R)*((2579692110316253*cos(q1R))/4503599627370496 - (1917820484151683*sin(q1R))/18014398509481984)) - (7514214926474921*sin(q3R)*(cos(q2R)*((2579692110316253*cos(q1R))/4503599627370496 - (1917820484151683*sin(q1R))/18014398509481984) - (32968958366167862000829996477285*sin(q2R))/40564819207303340847894502572032 + (7514214926474921*sin(q2R)*((1917820484151683*cos(q1R))/18014398509481984 + (2579692110316253*sin(q1R))/4503599627370496))/36893488147419103232))/36893488147419103232))/9007199254740992 - (3497003479222003021661409533057350838749300515155764632398442290070889008826875*sin(q2R))/509258994083621521567111422102344540262867098416484062659035112338595324940834176545849344 + (9007199067919185*((234819211581865*cos(q4R))/1152921504606846976 + (9007199067919185*sin(q4R))/9007199254740992)*((9007199067919185*cos(q2R)*((2579692110316253*cos(q1R))/4503599627370496 - (1917820484151683*sin(q1R))/18014398509481984))/9007199254740992 - (296957971066013582975066703729047659005068212725*sin(q2R))/365375409332725729550921208179070754913983135744 + (67682029681889335677290557259385*sin(q2R)*((1917820484151683*cos(q1R))/18014398509481984 + (2579692110316253*sin(q1R))/4503599627370496))/332306998946228968225951765070086144))/9007199254740992 + (1764482024691522628700660907665*cos(q3R)*((32968958366167862000829996477285*cos(q2R))/40564819207303340847894502572032 - (7514214926474921*cos(q2R)*((1917820484151683*cos(q1R))/18014398509481984 + (2579692110316253*sin(q1R))/4503599627370496))/36893488147419103232 + sin(q2R)*((2579692110316253*cos(q1R))/4503599627370496 - (1917820484151683*sin(q1R))/18014398509481984)))/42535295865117307932921825928971026432 + (508577317689771495245073589786522929324694383585*cos(q3R)*(cos(q2R)*((2579692110316253*cos(q1R))/4503599627370496 - (1917820484151683*sin(q1R))/18014398509481984) - (32968958366167862000829996477285*sin(q2R))/40564819207303340847894502572032 + (7514214926474921*sin(q2R)*((1917820484151683*cos(q1R))/18014398509481984 + (2579692110316253*sin(q1R))/4503599627370496))/36893488147419103232))/12259964326927110866866776217202473468949912977468817408 + (67682029681889335677290557259385*sin(q3R)*((32968958366167862000829996477285*cos(q2R))/40564819207303340847894502572032 - (7514214926474921*cos(q2R)*((1917820484151683*cos(q1R))/18014398509481984 + (2579692110316253*sin(q1R))/4503599627370496))/36893488147419103232 + sin(q2R)*((2579692110316253*cos(q1R))/4503599627370496 - (1917820484151683*sin(q1R))/18014398509481984)))/332306998946228968225951765070086144 - (13258697167433729449897784796786197386719169465*sin(q3R)*(cos(q2R)*((2579692110316253*cos(q1R))/4503599627370496 - (1917820484151683*sin(q1R))/18014398509481984) - (32968958366167862000829996477285*sin(q2R))/40564819207303340847894502572032 + (7514214926474921*sin(q2R)*((1917820484151683*cos(q1R))/18014398509481984 + (2579692110316253*sin(q1R))/4503599627370496))/36893488147419103232))/1569275433846670190958947355801916604025588861116008628224 - (67682029681889335677290557259385*cos(q4R)*((7514214926474921*cos(q3R)*(cos(q2R)*((2579692110316253*cos(q1R))/4503599627370496 - (1917820484151683*sin(q1R))/18014398509481984) - (32968958366167862000829996477285*sin(q2R))/40564819207303340847894502572032 + (7514214926474921*sin(q2R)*((1917820484151683*cos(q1R))/18014398509481984 + (2579692110316253*sin(q1R))/4503599627370496))/36893488147419103232))/36893488147419103232 + sin(q3R)*((32968958366167862000829996477285*cos(q2R))/40564819207303340847894502572032 - (7514214926474921*cos(q2R)*((1917820484151683*cos(q1R))/18014398509481984 + (2579692110316253*sin(q1R))/4503599627370496))/36893488147419103232 + sin(q2R)*((2579692110316253*cos(q1R))/4503599627370496 - (1917820484151683*sin(q1R))/18014398509481984))))/332306998946228968225951765070086144 + (106069577339469832923929692356850887620017617375*cos(q2R)*((2579692110316253*cos(q1R))/4503599627370496 - (1917820484151683*sin(q1R))/18014398509481984))/12554203470773361527671578846415332832204710888928069025792 + (797029601289130257223357069404502671534492977261568326111352375*sin(q2R)*((1917820484151683*cos(q1R))/18014398509481984 + (2579692110316253*sin(q1R))/4503599627370496))/463168356949264781694283940034751631413079938662562256157830336031652518559744))/16225927682921336339157801028812800 - (60617164743372705924380750591060836759586313939367162716784907429017787816377231*cos(q3R)*((32968958366167862000829996477285*cos(q2R))/40564819207303340847894502572032 - (7514214926474921*cos(q2R)*((1917820484151683*cos(q1R))/18014398509481984 + (2579692110316253*sin(q1R))/4503599627370496))/36893488147419103232 + sin(q2R)*((2579692110316253*cos(q1R))/4503599627370496 - (1917820484151683*sin(q1R))/18014398509481984)))/1447401115466452442794637312608598848165874808320507050493219800098914120499200000 - (324259171862923063*sin(q6R)*((7514214926474921*sin(q5R)*(((4503599440548691*cos(q4R))/4503599627370496 - (7514214926474921*sin(q4R))/36893488147419103232)*(cos(q3R)*((32968958366167862000829996477285*cos(q2R))/40564819207303340847894502572032 - (7514214926474921*cos(q2R)*((1917820484151683*cos(q1R))/18014398509481984 + (2579692110316253*sin(q1R))/4503599627370496))/36893488147419103232 + sin(q2R)*((2579692110316253*cos(q1R))/4503599627370496 - (1917820484151683*sin(q1R))/18014398509481984)) - (7514214926474921*sin(q3R)*(cos(q2R)*((2579692110316253*cos(q1R))/4503599627370496 - (1917820484151683*sin(q1R))/18014398509481984) - (32968958366167862000829996477285*sin(q2R))/40564819207303340847894502572032 + (7514214926474921*sin(q2R)*((1917820484151683*cos(q1R))/18014398509481984 + (2579692110316253*sin(q1R))/4503599627370496))/36893488147419103232))/36893488147419103232) + ((234819211581865*cos(q4R))/1152921504606846976 + (9007199067919185*sin(q4R))/9007199254740992)*((9007199067919185*cos(q2R)*((2579692110316253*cos(q1R))/4503599627370496 - (1917820484151683*sin(q1R))/18014398509481984))/9007199254740992 - (296957971066013582975066703729047659005068212725*sin(q2R))/365375409332725729550921208179070754913983135744 + (67682029681889335677290557259385*sin(q2R)*((1917820484151683*cos(q1R))/18014398509481984 + (2579692110316253*sin(q1R))/4503599627370496))/332306998946228968225951765070086144) - (7514214926474921*cos(q4R)*((7514214926474921*cos(q3R)*(cos(q2R)*((2579692110316253*cos(q1R))/4503599627370496 - (1917820484151683*sin(q1R))/18014398509481984) - (32968958366167862000829996477285*sin(q2R))/40564819207303340847894502572032 + (7514214926474921*sin(q2R)*((1917820484151683*cos(q1R))/18014398509481984 + (2579692110316253*sin(q1R))/4503599627370496))/36893488147419103232))/36893488147419103232 + sin(q3R)*((32968958366167862000829996477285*cos(q2R))/40564819207303340847894502572032 - (7514214926474921*cos(q2R)*((1917820484151683*cos(q1R))/18014398509481984 + (2579692110316253*sin(q1R))/4503599627370496))/36893488147419103232 + sin(q2R)*((2579692110316253*cos(q1R))/4503599627370496 - (1917820484151683*sin(q1R))/18014398509481984))))/36893488147419103232))/36893488147419103232 - (9007199067919185*sin(q5R)*((234819211581865*cos(q3R)*((32968958366167862000829996477285*cos(q2R))/40564819207303340847894502572032 - (7514214926474921*cos(q2R)*((1917820484151683*cos(q1R))/18014398509481984 + (2579692110316253*sin(q1R))/4503599627370496))/36893488147419103232 + sin(q2R)*((2579692110316253*cos(q1R))/4503599627370496 - (1917820484151683*sin(q1R))/18014398509481984)))/1152921504606846976 - (465385075279251052437186083221547446448384963368966483726351875*sin(q2R))/13803492693581127574869511724554050904902217944340773110325048447598592 + (67682029681889335677290557259385*cos(q3R)*(cos(q2R)*((2579692110316253*cos(q1R))/4503599627370496 - (1917820484151683*sin(q1R))/18014398509481984) - (32968958366167862000829996477285*sin(q2R))/40564819207303340847894502572032 + (7514214926474921*sin(q2R)*((1917820484151683*cos(q1R))/18014398509481984 + (2579692110316253*sin(q1R))/4503599627370496))/36893488147419103232))/332306998946228968225951765070086144 + (9007199067919185*sin(q3R)*((32968958366167862000829996477285*cos(q2R))/40564819207303340847894502572032 - (7514214926474921*cos(q2R)*((1917820484151683*cos(q1R))/18014398509481984 + (2579692110316253*sin(q1R))/4503599627370496))/36893488147419103232 + sin(q2R)*((2579692110316253*cos(q1R))/4503599627370496 - (1917820484151683*sin(q1R))/18014398509481984)))/9007199254740992 - (1764482024691522628700660907665*sin(q3R)*(cos(q2R)*((2579692110316253*cos(q1R))/4503599627370496 - (1917820484151683*sin(q1R))/18014398509481984) - (32968958366167862000829996477285*sin(q2R))/40564819207303340847894502572032 + (7514214926474921*sin(q2R)*((1917820484151683*cos(q1R))/18014398509481984 + (2579692110316253*sin(q1R))/4503599627370496))/36893488147419103232))/42535295865117307932921825928971026432 + (14115856197532180673579726082375*cos(q2R)*((2579692110316253*cos(q1R))/4503599627370496 - (1917820484151683*sin(q1R))/18014398509481984))/340282366920938463463374607431768211456 + (106069577339469832923929692356850887620017617375*sin(q2R)*((1917820484151683*cos(q1R))/18014398509481984 + (2579692110316253*sin(q1R))/4503599627370496))/12554203470773361527671578846415332832204710888928069025792))/9007199254740992 + cos(q5R)*(((9007199067919185*cos(q4R))/9007199254740992 - (234819211581865*sin(q4R))/1152921504606846976)*((9007199067919185*cos(q2R)*((2579692110316253*cos(q1R))/4503599627370496 - (1917820484151683*sin(q1R))/18014398509481984))/9007199254740992 - (296957971066013582975066703729047659005068212725*sin(q2R))/365375409332725729550921208179070754913983135744 + (67682029681889335677290557259385*sin(q2R)*((1917820484151683*cos(q1R))/18014398509481984 + (2579692110316253*sin(q1R))/4503599627370496))/332306998946228968225951765070086144) - ((7514214926474921*cos(q4R))/36893488147419103232 + (4503599440548691*sin(q4R))/4503599627370496)*(cos(q3R)*((32968958366167862000829996477285*cos(q2R))/40564819207303340847894502572032 - (7514214926474921*cos(q2R)*((1917820484151683*cos(q1R))/18014398509481984 + (2579692110316253*sin(q1R))/4503599627370496))/36893488147419103232 + sin(q2R)*((2579692110316253*cos(q1R))/4503599627370496 - (1917820484151683*sin(q1R))/18014398509481984)) - (7514214926474921*sin(q3R)*(cos(q2R)*((2579692110316253*cos(q1R))/4503599627370496 - (1917820484151683*sin(q1R))/18014398509481984) - (32968958366167862000829996477285*sin(q2R))/40564819207303340847894502572032 + (7514214926474921*sin(q2R)*((1917820484151683*cos(q1R))/18014398509481984 + (2579692110316253*sin(q1R))/4503599627370496))/36893488147419103232))/36893488147419103232) + (7514214926474921*sin(q4R)*((7514214926474921*cos(q3R)*(cos(q2R)*((2579692110316253*cos(q1R))/4503599627370496 - (1917820484151683*sin(q1R))/18014398509481984) - (32968958366167862000829996477285*sin(q2R))/40564819207303340847894502572032 + (7514214926474921*sin(q2R)*((1917820484151683*cos(q1R))/18014398509481984 + (2579692110316253*sin(q1R))/4503599627370496))/36893488147419103232))/36893488147419103232 + sin(q3R)*((32968958366167862000829996477285*cos(q2R))/40564819207303340847894502572032 - (7514214926474921*cos(q2R)*((1917820484151683*cos(q1R))/18014398509481984 + (2579692110316253*sin(q1R))/4503599627370496))/36893488147419103232 + sin(q2R)*((2579692110316253*cos(q1R))/4503599627370496 - (1917820484151683*sin(q1R))/18014398509481984))))/36893488147419103232)))/9007199254740992000 - (48638874966763599*sin(q6R)*((9007199067919185*((4503599440548691*cos(q4R))/4503599627370496 - (7514214926474921*sin(q4R))/36893488147419103232)*(cos(q3R)*((32968958366167862000829996477285*cos(q2R))/40564819207303340847894502572032 - (7514214926474921*cos(q2R)*((1917820484151683*cos(q1R))/18014398509481984 + (2579692110316253*sin(q1R))/4503599627370496))/36893488147419103232 + sin(q2R)*((2579692110316253*cos(q1R))/4503599627370496 - (1917820484151683*sin(q1R))/18014398509481984)) - (7514214926474921*sin(q3R)*(cos(q2R)*((2579692110316253*cos(q1R))/4503599627370496 - (1917820484151683*sin(q1R))/18014398509481984) - (32968958366167862000829996477285*sin(q2R))/40564819207303340847894502572032 + (7514214926474921*sin(q2R)*((1917820484151683*cos(q1R))/18014398509481984 + (2579692110316253*sin(q1R))/4503599627370496))/36893488147419103232))/36893488147419103232))/9007199254740992 - (3497003479222003021661409533057350838749300515155764632398442290070889008826875*sin(q2R))/509258994083621521567111422102344540262867098416484062659035112338595324940834176545849344 + (9007199067919185*((234819211581865*cos(q4R))/1152921504606846976 + (9007199067919185*sin(q4R))/9007199254740992)*((9007199067919185*cos(q2R)*((2579692110316253*cos(q1R))/4503599627370496 - (1917820484151683*sin(q1R))/18014398509481984))/9007199254740992 - (296957971066013582975066703729047659005068212725*sin(q2R))/365375409332725729550921208179070754913983135744 + (67682029681889335677290557259385*sin(q2R)*((1917820484151683*cos(q1R))/18014398509481984 + (2579692110316253*sin(q1R))/4503599627370496))/332306998946228968225951765070086144))/9007199254740992 + (1764482024691522628700660907665*cos(q3R)*((32968958366167862000829996477285*cos(q2R))/40564819207303340847894502572032 - (7514214926474921*cos(q2R)*((1917820484151683*cos(q1R))/18014398509481984 + (2579692110316253*sin(q1R))/4503599627370496))/36893488147419103232 + sin(q2R)*((2579692110316253*cos(q1R))/4503599627370496 - (1917820484151683*sin(q1R))/18014398509481984)))/42535295865117307932921825928971026432 + (508577317689771495245073589786522929324694383585*cos(q3R)*(cos(q2R)*((2579692110316253*cos(q1R))/4503599627370496 - (1917820484151683*sin(q1R))/18014398509481984) - (32968958366167862000829996477285*sin(q2R))/40564819207303340847894502572032 + (7514214926474921*sin(q2R)*((1917820484151683*cos(q1R))/18014398509481984 + (2579692110316253*sin(q1R))/4503599627370496))/36893488147419103232))/12259964326927110866866776217202473468949912977468817408 + (67682029681889335677290557259385*sin(q3R)*((32968958366167862000829996477285*cos(q2R))/40564819207303340847894502572032 - (7514214926474921*cos(q2R)*((1917820484151683*cos(q1R))/18014398509481984 + (2579692110316253*sin(q1R))/4503599627370496))/36893488147419103232 + sin(q2R)*((2579692110316253*cos(q1R))/4503599627370496 - (1917820484151683*sin(q1R))/18014398509481984)))/332306998946228968225951765070086144 - (13258697167433729449897784796786197386719169465*sin(q3R)*(cos(q2R)*((2579692110316253*cos(q1R))/4503599627370496 - (1917820484151683*sin(q1R))/18014398509481984) - (32968958366167862000829996477285*sin(q2R))/40564819207303340847894502572032 + (7514214926474921*sin(q2R)*((1917820484151683*cos(q1R))/18014398509481984 + (2579692110316253*sin(q1R))/4503599627370496))/36893488147419103232))/1569275433846670190958947355801916604025588861116008628224 - (67682029681889335677290557259385*cos(q4R)*((7514214926474921*cos(q3R)*(cos(q2R)*((2579692110316253*cos(q1R))/4503599627370496 - (1917820484151683*sin(q1R))/18014398509481984) - (32968958366167862000829996477285*sin(q2R))/40564819207303340847894502572032 + (7514214926474921*sin(q2R)*((1917820484151683*cos(q1R))/18014398509481984 + (2579692110316253*sin(q1R))/4503599627370496))/36893488147419103232))/36893488147419103232 + sin(q3R)*((32968958366167862000829996477285*cos(q2R))/40564819207303340847894502572032 - (7514214926474921*cos(q2R)*((1917820484151683*cos(q1R))/18014398509481984 + (2579692110316253*sin(q1R))/4503599627370496))/36893488147419103232 + sin(q2R)*((2579692110316253*cos(q1R))/4503599627370496 - (1917820484151683*sin(q1R))/18014398509481984))))/332306998946228968225951765070086144 + (106069577339469832923929692356850887620017617375*cos(q2R)*((2579692110316253*cos(q1R))/4503599627370496 - (1917820484151683*sin(q1R))/18014398509481984))/12554203470773361527671578846415332832204710888928069025792 + (797029601289130257223357069404502671534492977261568326111352375*sin(q2R)*((1917820484151683*cos(q1R))/18014398509481984 + (2579692110316253*sin(q1R))/4503599627370496))/463168356949264781694283940034751631413079938662562256157830336031652518559744))/1801439850948198400 - (347469655025336708709976918716104493695816557877713443586884917071777956519687017125887603*cos(q3R)*(cos(q2R)*((2579692110316253*cos(q1R))/4503599627370496 - (1917820484151683*sin(q1R))/18014398509481984) - (32968958366167862000829996477285*sin(q2R))/40564819207303340847894502572032 + (7514214926474921*sin(q2R)*((1917820484151683*cos(q1R))/18014398509481984 + (2579692110316253*sin(q1R))/4503599627370496))/36893488147419103232))/83436993590660550093555535397248129476668145404556748826056312805555458038306271485271956520960000 - (46241644459901303158631016767207157814229090534989303509431886332469146043*sin(q3R)*((32968958366167862000829996477285*cos(q2R))/40564819207303340847894502572032 - (7514214926474921*cos(q2R)*((1917820484151683*cos(q1R))/18014398509481984 + (2579692110316253*sin(q1R))/4503599627370496))/36893488147419103232 + sin(q2R)*((2579692110316253*cos(q1R))/4503599627370496 - (1917820484151683*sin(q1R))/18014398509481984)))/2261564242916331941866620800950935700259179388000792266395655937654553313280000 + (455490404115240510935077772268745492204390157443214084883134054419271951750419293234291596923751*sin(q3R)*(cos(q2R)*((2579692110316253*cos(q1R))/4503599627370496 - (1917820484151683*sin(q1R))/18014398509481984) - (32968958366167862000829996477285*sin(q2R))/40564819207303340847894502572032 + (7514214926474921*sin(q2R)*((1917820484151683*cos(q1R))/18014398509481984 + (2579692110316253*sin(q1R))/4503599627370496))/36893488147419103232))/53399675898022752059875542654238802865067613058916319248676040195555493144516013750574052173414400000 + (610321541873521657855151997354401418608858870661075444886782706002880706727*cos(q4R)*((7514214926474921*cos(q3R)*(cos(q2R)*((2579692110316253*cos(q1R))/4503599627370496 - (1917820484151683*sin(q1R))/18014398509481984) - (32968958366167862000829996477285*sin(q2R))/40564819207303340847894502572032 + (7514214926474921*sin(q2R)*((1917820484151683*cos(q1R))/18014398509481984 + (2579692110316253*sin(q1R))/4503599627370496))/36893488147419103232))/36893488147419103232 + sin(q3R)*((32968958366167862000829996477285*cos(q2R))/40564819207303340847894502572032 - (7514214926474921*cos(q2R)*((1917820484151683*cos(q1R))/18014398509481984 + (2579692110316253*sin(q1R))/4503599627370496))/36893488147419103232 + sin(q2R)*((2579692110316253*cos(q1R))/4503599627370496 - (1917820484151683*sin(q1R))/18014398509481984))))/11307821214581659709333104004754678501295896940003961331978279688272766566400000 + (608651409044468601*sin(q4R)*((7514214926474921*cos(q3R)*(cos(q2R)*((2579692110316253*cos(q1R))/4503599627370496 - (1917820484151683*sin(q1R))/18014398509481984) - (32968958366167862000829996477285*sin(q2R))/40564819207303340847894502572032 + (7514214926474921*sin(q2R)*((1917820484151683*cos(q1R))/18014398509481984 + (2579692110316253*sin(q1R))/4503599627370496))/36893488147419103232))/36893488147419103232 + sin(q3R)*((32968958366167862000829996477285*cos(q2R))/40564819207303340847894502572032 - (7514214926474921*cos(q2R)*((1917820484151683*cos(q1R))/18014398509481984 + (2579692110316253*sin(q1R))/4503599627370496))/36893488147419103232 + sin(q2R)*((2579692110316253*cos(q1R))/4503599627370496 - (1917820484151683*sin(q1R))/18014398509481984))))/73786976294838206464000 + (107465779053290185796889472867275736954369330186921663479979246519176992895505610212310958309481948671*cos(q2R)*((2579692110316253*cos(q1R))/4503599627370496 - (1917820484151683*sin(q1R))/18014398509481984))/427197407184182016479004341233910422920540904471330553989408321564443945156128110004592417387315200000 + (22542644779424763*cos(q2R)*((1917820484151683*cos(q1R))/18014398509481984 + (2579692110316253*sin(q1R))/4503599627370496))/3689348814741910323200 - (3*sin(q2R)*((2579692110316253*cos(q1R))/4503599627370496 - (1917820484151683*sin(q1R))/18014398509481984))/100 + (807520961047489018778067709720399904923771262077295170375712179706208528987338271217011451790113918662491539890779991*sin(q2R)*((1917820484151683*cos(q1R))/18014398509481984 + (2579692110316253*sin(q1R))/4503599627370496))/15760802478557791684911616040057445522031895708186178667179317361698288708598884244565706501953966256322651196122726400000 - (170695144106365826517608855445768431563113584343*cos(q5R)*((234819211581865*cos(q3R)*((32968958366167862000829996477285*cos(q2R))/40564819207303340847894502572032 - (7514214926474921*cos(q2R)*((1917820484151683*cos(q1R))/18014398509481984 + (2579692110316253*sin(q1R))/4503599627370496))/36893488147419103232 + sin(q2R)*((2579692110316253*cos(q1R))/4503599627370496 - (1917820484151683*sin(q1R))/18014398509481984)))/1152921504606846976 - (465385075279251052437186083221547446448384963368966483726351875*sin(q2R))/13803492693581127574869511724554050904902217944340773110325048447598592 + (67682029681889335677290557259385*cos(q3R)*(cos(q2R)*((2579692110316253*cos(q1R))/4503599627370496 - (1917820484151683*sin(q1R))/18014398509481984) - (32968958366167862000829996477285*sin(q2R))/40564819207303340847894502572032 + (7514214926474921*sin(q2R)*((1917820484151683*cos(q1R))/18014398509481984 + (2579692110316253*sin(q1R))/4503599627370496))/36893488147419103232))/332306998946228968225951765070086144 + (9007199067919185*sin(q3R)*((32968958366167862000829996477285*cos(q2R))/40564819207303340847894502572032 - (7514214926474921*cos(q2R)*((1917820484151683*cos(q1R))/18014398509481984 + (2579692110316253*sin(q1R))/4503599627370496))/36893488147419103232 + sin(q2R)*((2579692110316253*cos(q1R))/4503599627370496 - (1917820484151683*sin(q1R))/18014398509481984)))/9007199254740992 - (1764482024691522628700660907665*sin(q3R)*(cos(q2R)*((2579692110316253*cos(q1R))/4503599627370496 - (1917820484151683*sin(q1R))/18014398509481984) - (32968958366167862000829996477285*sin(q2R))/40564819207303340847894502572032 + (7514214926474921*sin(q2R)*((1917820484151683*cos(q1R))/18014398509481984 + (2579692110316253*sin(q1R))/4503599627370496))/36893488147419103232))/42535295865117307932921825928971026432 + (14115856197532180673579726082375*cos(q2R)*((2579692110316253*cos(q1R))/4503599627370496 - (1917820484151683*sin(q1R))/18014398509481984))/340282366920938463463374607431768211456 + (106069577339469832923929692356850887620017617375*sin(q2R)*((1917820484151683*cos(q1R))/18014398509481984 + (2579692110316253*sin(q1R))/4503599627370496))/12554203470773361527671578846415332832204710888928069025792))/119726214130147567059245861496117904970213993920593920, (27*cos(q5R)*(((7514214926474921*cos(q4R))/36893488147419103232 + (4503599440548691*sin(q4R))/4503599627370496)*((9007199067919185*cos(q3R)*((17274190877287359225804725738355*cos(q1R))/162259276829213363391578010288128 + (23235800371559029388956996013805*sin(q1R))/40564819207303340847894502572032 + 27504203825998033884751021716381/166153499473114484112975882535043072))/9007199254740992 - (7514214926474921*cos(q3R)*((32968958366167862000829996477285*cos(q2R))/40564819207303340847894502572032 - (7514214926474921*cos(q2R)*((1917820484151683*cos(q1R))/18014398509481984 + (2579692110316253*sin(q1R))/4503599627370496))/36893488147419103232 + sin(q2R)*((2579692110316253*cos(q1R))/4503599627370496 - (1917820484151683*sin(q1R))/18014398509481984)))/36893488147419103232 + sin(q3R)*(cos(q2R)*((2579692110316253*cos(q1R))/4503599627370496 - (1917820484151683*sin(q1R))/18014398509481984) - (32968958366167862000829996477285*sin(q2R))/40564819207303340847894502572032 + (7514214926474921*sin(q2R)*((1917820484151683*cos(q1R))/18014398509481984 + (2579692110316253*sin(q1R))/4503599627370496))/36893488147419103232)) + (7514214926474921*sin(q4R)*(cos(q3R)*(cos(q2R)*((2579692110316253*cos(q1R))/4503599627370496 - (1917820484151683*sin(q1R))/18014398509481984) - (32968958366167862000829996477285*sin(q2R))/40564819207303340847894502572032 + (7514214926474921*sin(q2R)*((1917820484151683*cos(q1R))/18014398509481984 + (2579692110316253*sin(q1R))/4503599627370496))/36893488147419103232) - (9007199067919185*sin(q3R)*((17274190877287359225804725738355*cos(q1R))/162259276829213363391578010288128 + (23235800371559029388956996013805*sin(q1R))/40564819207303340847894502572032 + 27504203825998033884751021716381/166153499473114484112975882535043072))/9007199254740992 + (7514214926474921*sin(q3R)*((32968958366167862000829996477285*cos(q2R))/40564819207303340847894502572032 - (7514214926474921*cos(q2R)*((1917820484151683*cos(q1R))/18014398509481984 + (2579692110316253*sin(q1R))/4503599627370496))/36893488147419103232 + sin(q2R)*((2579692110316253*cos(q1R))/4503599627370496 - (1917820484151683*sin(q1R))/18014398509481984)))/36893488147419103232))/36893488147419103232))/1000 - (202883803014822867*sin(q5R)*(((4503599440548691*cos(q4R))/4503599627370496 - (7514214926474921*sin(q4R))/36893488147419103232)*((9007199067919185*cos(q3R)*((17274190877287359225804725738355*cos(q1R))/162259276829213363391578010288128 + (23235800371559029388956996013805*sin(q1R))/40564819207303340847894502572032 + 27504203825998033884751021716381/166153499473114484112975882535043072))/9007199254740992 - (7514214926474921*cos(q3R)*((32968958366167862000829996477285*cos(q2R))/40564819207303340847894502572032 - (7514214926474921*cos(q2R)*((1917820484151683*cos(q1R))/18014398509481984 + (2579692110316253*sin(q1R))/4503599627370496))/36893488147419103232 + sin(q2R)*((2579692110316253*cos(q1R))/4503599627370496 - (1917820484151683*sin(q1R))/18014398509481984)))/36893488147419103232 + sin(q3R)*(cos(q2R)*((2579692110316253*cos(q1R))/4503599627370496 - (1917820484151683*sin(q1R))/18014398509481984) - (32968958366167862000829996477285*sin(q2R))/40564819207303340847894502572032 + (7514214926474921*sin(q2R)*((1917820484151683*cos(q1R))/18014398509481984 + (2579692110316253*sin(q1R))/4503599627370496))/36893488147419103232)) + (7514214926474921*cos(q4R)*(cos(q3R)*(cos(q2R)*((2579692110316253*cos(q1R))/4503599627370496 - (1917820484151683*sin(q1R))/18014398509481984) - (32968958366167862000829996477285*sin(q2R))/40564819207303340847894502572032 + (7514214926474921*sin(q2R)*((1917820484151683*cos(q1R))/18014398509481984 + (2579692110316253*sin(q1R))/4503599627370496))/36893488147419103232) - (9007199067919185*sin(q3R)*((17274190877287359225804725738355*cos(q1R))/162259276829213363391578010288128 + (23235800371559029388956996013805*sin(q1R))/40564819207303340847894502572032 + 27504203825998033884751021716381/166153499473114484112975882535043072))/9007199254740992 + (7514214926474921*sin(q3R)*((32968958366167862000829996477285*cos(q2R))/40564819207303340847894502572032 - (7514214926474921*cos(q2R)*((1917820484151683*cos(q1R))/18014398509481984 + (2579692110316253*sin(q1R))/4503599627370496))/36893488147419103232 + sin(q2R)*((2579692110316253*cos(q1R))/4503599627370496 - (1917820484151683*sin(q1R))/18014398509481984)))/36893488147419103232))/36893488147419103232))/36893488147419103232000 - (109198173955282063961996941994332957526645881091499469714283881779231664456243735535448036415347*cos(q3R)*((17274190877287359225804725738355*cos(q1R))/162259276829213363391578010288128 + (23235800371559029388956996013805*sin(q1R))/40564819207303340847894502572032 + 27504203825998033884751021716381/166153499473114484112975882535043072))/2607406049708142190423610481164004046145879543892398400814259775173608063697070983914748641280000 + (94754841554645069948206780163139*sin(q5R)*(((7514214926474921*cos(q4R))/36893488147419103232 + (4503599440548691*sin(q4R))/4503599627370496)*((9007199067919185*cos(q3R)*((17274190877287359225804725738355*cos(q1R))/162259276829213363391578010288128 + (23235800371559029388956996013805*sin(q1R))/40564819207303340847894502572032 + 27504203825998033884751021716381/166153499473114484112975882535043072))/9007199254740992 - (7514214926474921*cos(q3R)*((32968958366167862000829996477285*cos(q2R))/40564819207303340847894502572032 - (7514214926474921*cos(q2R)*((1917820484151683*cos(q1R))/18014398509481984 + (2579692110316253*sin(q1R))/4503599627370496))/36893488147419103232 + sin(q2R)*((2579692110316253*cos(q1R))/4503599627370496 - (1917820484151683*sin(q1R))/18014398509481984)))/36893488147419103232 + sin(q3R)*(cos(q2R)*((2579692110316253*cos(q1R))/4503599627370496 - (1917820484151683*sin(q1R))/18014398509481984) - (32968958366167862000829996477285*sin(q2R))/40564819207303340847894502572032 + (7514214926474921*sin(q2R)*((1917820484151683*cos(q1R))/18014398509481984 + (2579692110316253*sin(q1R))/4503599627370496))/36893488147419103232)) + (7514214926474921*sin(q4R)*(cos(q3R)*(cos(q2R)*((2579692110316253*cos(q1R))/4503599627370496 - (1917820484151683*sin(q1R))/18014398509481984) - (32968958366167862000829996477285*sin(q2R))/40564819207303340847894502572032 + (7514214926474921*sin(q2R)*((1917820484151683*cos(q1R))/18014398509481984 + (2579692110316253*sin(q1R))/4503599627370496))/36893488147419103232) - (9007199067919185*sin(q3R)*((17274190877287359225804725738355*cos(q1R))/162259276829213363391578010288128 + (23235800371559029388956996013805*sin(q1R))/40564819207303340847894502572032 + 27504203825998033884751021716381/166153499473114484112975882535043072))/9007199254740992 + (7514214926474921*sin(q3R)*((32968958366167862000829996477285*cos(q2R))/40564819207303340847894502572032 - (7514214926474921*cos(q2R)*((1917820484151683*cos(q1R))/18014398509481984 + (2579692110316253*sin(q1R))/4503599627370496))/36893488147419103232 + sin(q2R)*((2579692110316253*cos(q1R))/4503599627370496 - (1917820484151683*sin(q1R))/18014398509481984)))/36893488147419103232))/36893488147419103232))/66461399789245793645190353014017228800 - (83301539375654672537075965313343183841442266989297270401707771044036658496661398777306991*sin(q3R)*((17274190877287359225804725738355*cos(q1R))/162259276829213363391578010288128 + (23235800371559029388956996013805*sin(q1R))/40564819207303340847894502572032 + 27504203825998033884751021716381/166153499473114484112975882535043072))/4074071952668972172536891376818756322102936787331872501272280898708762599526673412366794752000 - (81222263116692158804177042061221826384594597321566869716687*((4503599440548691*cos(q4R))/4503599627370496 - (7514214926474921*sin(q4R))/36893488147419103232)*((9007199067919185*cos(q3R)*((17274190877287359225804725738355*cos(q1R))/162259276829213363391578010288128 + (23235800371559029388956996013805*sin(q1R))/40564819207303340847894502572032 + 27504203825998033884751021716381/166153499473114484112975882535043072))/9007199254740992 - (7514214926474921*cos(q3R)*((32968958366167862000829996477285*cos(q2R))/40564819207303340847894502572032 - (7514214926474921*cos(q2R)*((1917820484151683*cos(q1R))/18014398509481984 + (2579692110316253*sin(q1R))/4503599627370496))/36893488147419103232 + sin(q2R)*((2579692110316253*cos(q1R))/4503599627370496 - (1917820484151683*sin(q1R))/18014398509481984)))/36893488147419103232 + sin(q3R)*(cos(q2R)*((2579692110316253*cos(q1R))/4503599627370496 - (1917820484151683*sin(q1R))/18014398509481984) - (32968958366167862000829996477285*sin(q2R))/40564819207303340847894502572032 + (7514214926474921*sin(q2R)*((1917820484151683*cos(q1R))/18014398509481984 + (2579692110316253*sin(q1R))/4503599627370496))/36893488147419103232)))/306499108173177771671669405430061836723747824436720435200000 - (81*((7514214926474921*cos(q4R))/36893488147419103232 + (4503599440548691*sin(q4R))/4503599627370496)*((9007199067919185*cos(q3R)*((17274190877287359225804725738355*cos(q1R))/162259276829213363391578010288128 + (23235800371559029388956996013805*sin(q1R))/40564819207303340847894502572032 + 27504203825998033884751021716381/166153499473114484112975882535043072))/9007199254740992 - (7514214926474921*cos(q3R)*((32968958366167862000829996477285*cos(q2R))/40564819207303340847894502572032 - (7514214926474921*cos(q2R)*((1917820484151683*cos(q1R))/18014398509481984 + (2579692110316253*sin(q1R))/4503599627370496))/36893488147419103232 + sin(q2R)*((2579692110316253*cos(q1R))/4503599627370496 - (1917820484151683*sin(q1R))/18014398509481984)))/36893488147419103232 + sin(q3R)*(cos(q2R)*((2579692110316253*cos(q1R))/4503599627370496 - (1917820484151683*sin(q1R))/18014398509481984) - (32968958366167862000829996477285*sin(q2R))/40564819207303340847894502572032 + (7514214926474921*sin(q2R)*((1917820484151683*cos(q1R))/18014398509481984 + (2579692110316253*sin(q1R))/4503599627370496))/36893488147419103232)))/2000 + (455490404115240510935077772268745492204390157443214084883134054419271951750419293234291596923751*cos(q3R)*((32968958366167862000829996477285*cos(q2R))/40564819207303340847894502572032 - (7514214926474921*cos(q2R)*((1917820484151683*cos(q1R))/18014398509481984 + (2579692110316253*sin(q1R))/4503599627370496))/36893488147419103232 + sin(q2R)*((2579692110316253*cos(q1R))/4503599627370496 - (1917820484151683*sin(q1R))/18014398509481984)))/53399675898022752059875542654238802865067613058916319248676040195555493144516013750574052173414400000 + (46241644459901303158631016767207157814229090534989303509431886332469146043*cos(q3R)*(cos(q2R)*((2579692110316253*cos(q1R))/4503599627370496 - (1917820484151683*sin(q1R))/18014398509481984) - (32968958366167862000829996477285*sin(q2R))/40564819207303340847894502572032 + (7514214926474921*sin(q2R)*((1917820484151683*cos(q1R))/18014398509481984 + (2579692110316253*sin(q1R))/4503599627370496))/36893488147419103232))/2261564242916331941866620800950935700259179388000792266395655937654553313280000 + (347469655025336708709976918716104493695816557877713443586884917071777956519687017125887603*sin(q3R)*((32968958366167862000829996477285*cos(q2R))/40564819207303340847894502572032 - (7514214926474921*cos(q2R)*((1917820484151683*cos(q1R))/18014398509481984 + (2579692110316253*sin(q1R))/4503599627370496))/36893488147419103232 + sin(q2R)*((2579692110316253*cos(q1R))/4503599627370496 - (1917820484151683*sin(q1R))/18014398509481984)))/83436993590660550093555535397248129476668145404556748826056312805555458038306271485271956520960000 - (60617164743372705924380750591060836759586313939367162716784907429017787816377231*sin(q3R)*(cos(q2R)*((2579692110316253*cos(q1R))/4503599627370496 - (1917820484151683*sin(q1R))/18014398509481984) - (32968958366167862000829996477285*sin(q2R))/40564819207303340847894502572032 + (7514214926474921*sin(q2R)*((1917820484151683*cos(q1R))/18014398509481984 + (2579692110316253*sin(q1R))/4503599627370496))/36893488147419103232))/1447401115466452442794637312608598848165874808320507050493219800098914120499200000 - (170695144106365826517608855445768431563113584343*cos(q5R)*((2115063383689692319117831580025*cos(q3R)*((17274190877287359225804725738355*cos(q1R))/162259276829213363391578010288128 + (23235800371559029388956996013805*sin(q1R))/40564819207303340847894502572032 + 27504203825998033884751021716381/166153499473114484112975882535043072))/10384593717069655257060992658440192 + (81129635049124235038645691064225*sin(q3R)*((17274190877287359225804725738355*cos(q1R))/162259276829213363391578010288128 + (23235800371559029388956996013805*sin(q1R))/40564819207303340847894502572032 + 27504203825998033884751021716381/166153499473114484112975882535043072))/81129638414606681695789005144064 - (1764482024691522628700660907665*cos(q3R)*((32968958366167862000829996477285*cos(q2R))/40564819207303340847894502572032 - (7514214926474921*cos(q2R)*((1917820484151683*cos(q1R))/18014398509481984 + (2579692110316253*sin(q1R))/4503599627370496))/36893488147419103232 + sin(q2R)*((2579692110316253*cos(q1R))/4503599627370496 - (1917820484151683*sin(q1R))/18014398509481984)))/42535295865117307932921825928971026432 - (9007199067919185*cos(q3R)*(cos(q2R)*((2579692110316253*cos(q1R))/4503599627370496 - (1917820484151683*sin(q1R))/18014398509481984) - (32968958366167862000829996477285*sin(q2R))/40564819207303340847894502572032 + (7514214926474921*sin(q2R)*((1917820484151683*cos(q1R))/18014398509481984 + (2579692110316253*sin(q1R))/4503599627370496))/36893488147419103232))/9007199254740992 - (67682029681889335677290557259385*sin(q3R)*((32968958366167862000829996477285*cos(q2R))/40564819207303340847894502572032 - (7514214926474921*cos(q2R)*((1917820484151683*cos(q1R))/18014398509481984 + (2579692110316253*sin(q1R))/4503599627370496))/36893488147419103232 + sin(q2R)*((2579692110316253*cos(q1R))/4503599627370496 - (1917820484151683*sin(q1R))/18014398509481984)))/332306998946228968225951765070086144 + (234819211581865*sin(q3R)*(cos(q2R)*((2579692110316253*cos(q1R))/4503599627370496 - (1917820484151683*sin(q1R))/18014398509481984) - (32968958366167862000829996477285*sin(q2R))/40564819207303340847894502572032 + (7514214926474921*sin(q2R)*((1917820484151683*cos(q1R))/18014398509481984 + (2579692110316253*sin(q1R))/4503599627370496))/36893488147419103232))/1152921504606846976))/119726214130147567059245861496117904970213993920593920 + (48638874966763599*sin(q5R)*((2115063383689692319117831580025*cos(q3R)*((17274190877287359225804725738355*cos(q1R))/162259276829213363391578010288128 + (23235800371559029388956996013805*sin(q1R))/40564819207303340847894502572032 + 27504203825998033884751021716381/166153499473114484112975882535043072))/10384593717069655257060992658440192 + (81129635049124235038645691064225*sin(q3R)*((17274190877287359225804725738355*cos(q1R))/162259276829213363391578010288128 + (23235800371559029388956996013805*sin(q1R))/40564819207303340847894502572032 + 27504203825998033884751021716381/166153499473114484112975882535043072))/81129638414606681695789005144064 - (1764482024691522628700660907665*cos(q3R)*((32968958366167862000829996477285*cos(q2R))/40564819207303340847894502572032 - (7514214926474921*cos(q2R)*((1917820484151683*cos(q1R))/18014398509481984 + (2579692110316253*sin(q1R))/4503599627370496))/36893488147419103232 + sin(q2R)*((2579692110316253*cos(q1R))/4503599627370496 - (1917820484151683*sin(q1R))/18014398509481984)))/42535295865117307932921825928971026432 - (9007199067919185*cos(q3R)*(cos(q2R)*((2579692110316253*cos(q1R))/4503599627370496 - (1917820484151683*sin(q1R))/18014398509481984) - (32968958366167862000829996477285*sin(q2R))/40564819207303340847894502572032 + (7514214926474921*sin(q2R)*((1917820484151683*cos(q1R))/18014398509481984 + (2579692110316253*sin(q1R))/4503599627370496))/36893488147419103232))/9007199254740992 - (67682029681889335677290557259385*sin(q3R)*((32968958366167862000829996477285*cos(q2R))/40564819207303340847894502572032 - (7514214926474921*cos(q2R)*((1917820484151683*cos(q1R))/18014398509481984 + (2579692110316253*sin(q1R))/4503599627370496))/36893488147419103232 + sin(q2R)*((2579692110316253*cos(q1R))/4503599627370496 - (1917820484151683*sin(q1R))/18014398509481984)))/332306998946228968225951765070086144 + (234819211581865*sin(q3R)*(cos(q2R)*((2579692110316253*cos(q1R))/4503599627370496 - (1917820484151683*sin(q1R))/18014398509481984) - (32968958366167862000829996477285*sin(q2R))/40564819207303340847894502572032 + (7514214926474921*sin(q2R)*((1917820484151683*cos(q1R))/18014398509481984 + (2579692110316253*sin(q1R))/4503599627370496))/36893488147419103232))/1152921504606846976))/1801439850948198400 - (584133382113593486367040631332731*cos(q6R)*((15893040848161638993908057577265778144967053025*cos(q3R)*((17274190877287359225804725738355*cos(q1R))/162259276829213363391578010288128 + (23235800371559029388956996013805*sin(q1R))/40564819207303340847894502572032 + 27504203825998033884751021716381/166153499473114484112975882535043072))/383123885216472214589586756787577295904684780545900544 + (609625514665592237562888769449172969868262801225*sin(q3R)*((17274190877287359225804725738355*cos(q1R))/162259276829213363391578010288128 + (23235800371559029388956996013805*sin(q1R))/40564819207303340847894502572032 + 27504203825998033884751021716381/166153499473114484112975882535043072))/2993155353253689176481146537402947624255349848014848 + (9007199067919185*((4503599440548691*cos(q4R))/4503599627370496 - (7514214926474921*sin(q4R))/36893488147419103232)*((9007199067919185*cos(q3R)*((17274190877287359225804725738355*cos(q1R))/162259276829213363391578010288128 + (23235800371559029388956996013805*sin(q1R))/40564819207303340847894502572032 + 27504203825998033884751021716381/166153499473114484112975882535043072))/9007199254740992 - (7514214926474921*cos(q3R)*((32968958366167862000829996477285*cos(q2R))/40564819207303340847894502572032 - (7514214926474921*cos(q2R)*((1917820484151683*cos(q1R))/18014398509481984 + (2579692110316253*sin(q1R))/4503599627370496))/36893488147419103232 + sin(q2R)*((2579692110316253*cos(q1R))/4503599627370496 - (1917820484151683*sin(q1R))/18014398509481984)))/36893488147419103232 + sin(q3R)*(cos(q2R)*((2579692110316253*cos(q1R))/4503599627370496 - (1917820484151683*sin(q1R))/18014398509481984) - (32968958366167862000829996477285*sin(q2R))/40564819207303340847894502572032 + (7514214926474921*sin(q2R)*((1917820484151683*cos(q1R))/18014398509481984 + (2579692110316253*sin(q1R))/4503599627370496))/36893488147419103232)))/9007199254740992 - (13258697167433729449897784796786197386719169465*cos(q3R)*((32968958366167862000829996477285*cos(q2R))/40564819207303340847894502572032 - (7514214926474921*cos(q2R)*((1917820484151683*cos(q1R))/18014398509481984 + (2579692110316253*sin(q1R))/4503599627370496))/36893488147419103232 + sin(q2R)*((2579692110316253*cos(q1R))/4503599627370496 - (1917820484151683*sin(q1R))/18014398509481984)))/1569275433846670190958947355801916604025588861116008628224 - (67682029681889335677290557259385*cos(q3R)*(cos(q2R)*((2579692110316253*cos(q1R))/4503599627370496 - (1917820484151683*sin(q1R))/18014398509481984) - (32968958366167862000829996477285*sin(q2R))/40564819207303340847894502572032 + (7514214926474921*sin(q2R)*((1917820484151683*cos(q1R))/18014398509481984 + (2579692110316253*sin(q1R))/4503599627370496))/36893488147419103232))/332306998946228968225951765070086144 - (508577317689771495245073589786522929324694383585*sin(q3R)*((32968958366167862000829996477285*cos(q2R))/40564819207303340847894502572032 - (7514214926474921*cos(q2R)*((1917820484151683*cos(q1R))/18014398509481984 + 